simulink model "DiagCCaller_TestHarness"  (R2019a)
settings: Solver=FixedStepDiscrete  StartTime=0.0  StopTime=10.0  FixedStep=0.1  RelTol=1e-3  EnableMultiTasking=on
undefined symbols (not defined in the file): Dem_EventStatusType, sigbuilder_block
(part 3 of 4)

== system DiagCCaller_TestHarness/Fault set and recover , FaultCnt = 10, PassCnt = -5 , Heal =1, JumpDownEn = 0  ==
  Bus Creator : BusCreator  Inputs=15
  Data Type Conversion{,1..2,9..14} (9 alike) : DataTypeConversion  OutDataTypeStr=boolean
  Data Type Conversion3 : DataTypeConversion  OutDataTypeStr=single
  Data Type Conversion4 : DataTypeConversion  OutDataTypeStr=single
  Data Type Conversion{5..8} (4 alike) : DataTypeConversion  OutDataTypeStr=int16
  Signal Builder : Subsystem  Tag=STV Subsys  LoadFcn=sigbuilder_block('load');  StartFcn=sigbuilder_block('start');  StopFcn=sigbuilder_block('stop');  ClipboardFcn=sigbuilder_block('clipboard');  TreatAsAtomicUnit=on  mask(Sigbuilder block){tuvar=[0:10]}
      mask help: Simulink:masks:SigbuilderBlock_MD
      mask init:
      | if ~strcmp(get_param(bdroot(gcbh),'SimulationStatus'),'stopped') tuvar = sigbuilder_block('maskInit'); end
      settings: CopyFcn=sigbuilder_block('copy');  DeleteFcn=sigbuilder_block('delete');  ModelCloseFcn=sigbuilder_block('modelClose');  PreSaveFcn=sigbuilder_block('preSave');  PauseFcn=sigbuilder_block('pause');  ContinueFcn=sigbuilder_block('continue');  NameChangeFcn=sigbuilder_block('namechange');  OpenFcn=sigbuilder_block('open',[5.4 30 1141.2 522.6 ]);  CloseFcn=sigbuilder_block('close');
      mask Display: plot(0, 0, 100, 100,[2, 2, 32, 32, 2], [68, 8, 8, 68, 68],[32, 2], [38, 38], [32, 19, 2],[53, 60, 44], [32, 17, 17, 2],[16, 16, 31, 31]);txt = getActiveGroup(gcbh);text(2, 100, txt,'verticalAlignment', 'top');
  Out1 : Outport
  wires:
  Bus Creator/1 -> Out1/1
  Signal Builder/2(DiagInput) -> Data Type Conversion1/1
  Signal Builder/3(StartupComp) -> Data Type Conversion2/1
  Signal Builder/4(MaxValue) -> Data Type Conversion4/1
  Signal Builder/5(MinValue) -> Data Type Conversion3/1
  Signal Builder/6(UpCount) -> Data Type Conversion5/1
  Signal Builder/7(DownCount) -> Data Type Conversion6/1
  Signal Builder/8(FaultCountThd) -> Data Type Conversion7/1
  Signal Builder/9(PassCountThd) -> Data Type Conversion8/1
  Signal Builder/10(DebounceEn) -> Data Type Conversion9/1
  Signal Builder/11(DiagReset) -> Data Type Conversion10/1
  Signal Builder/12(DiagEnable) -> Data Type Conversion11/1
  Signal Builder/13(HealEnable) -> Data Type Conversion12/1
  Signal Builder/14(PreestorageFreezeTrigger) -> Data Type Conversion13/1
  Signal Builder/15(JumpDownEn) -> Data Type Conversion14/1
  Signal Builder/1(EnableSubsystem) -> Data Type Conversion/1
  Data Type Conversion/1 -> Bus Creator/1  "EnableSubsystem"
  Data Type Conversion1/1 -> Bus Creator/2  "DiagInput"
  Data Type Conversion2/1 -> Bus Creator/3  "StartupComp"
  Data Type Conversion4/1 -> Bus Creator/4  "MaxValue"
  Data Type Conversion3/1 -> Bus Creator/5  "MinValue"
  Data Type Conversion5/1 -> Bus Creator/6  "UpCount"
  Data Type Conversion6/1 -> Bus Creator/7  "DownCount"
  Data Type Conversion7/1 -> Bus Creator/8  "FaultCountThd"
  Data Type Conversion8/1 -> Bus Creator/9  "PassCountThd"
  Data Type Conversion9/1 -> Bus Creator/10  "DebounceEn"
  Data Type Conversion10/1 -> Bus Creator/11  "DiagReset"
  Data Type Conversion11/1 -> Bus Creator/12  "DiagEnable"
  Data Type Conversion12/1 -> Bus Creator/13  "HealEnable"
  Data Type Conversion13/1 -> Bus Creator/14  "PreestorageFreezeTrigger"
  Data Type Conversion14/1 -> Bus Creator/15  "JumpDownEn"

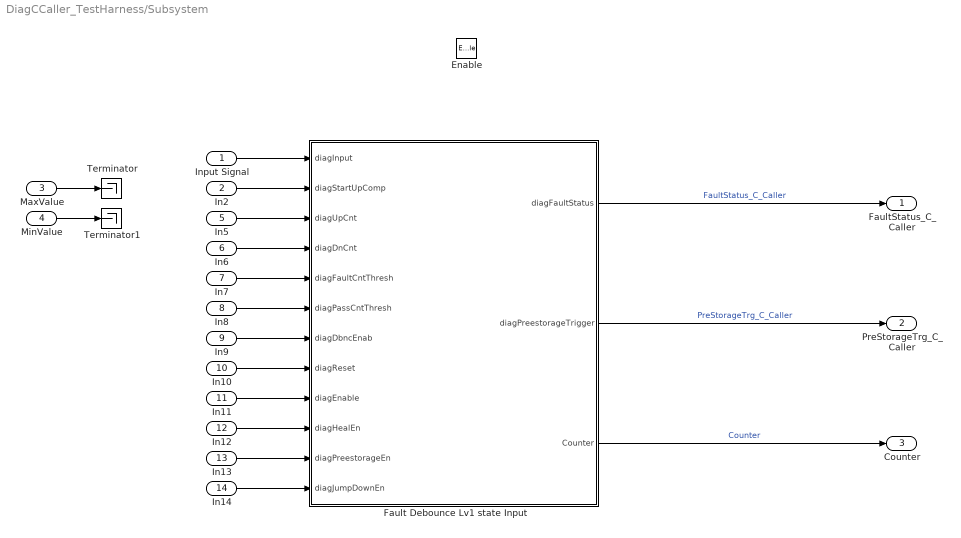
== system DiagCCaller_TestHarness/Subsystem ==
  Input Signal : Inport
  In2 : Inport  Port=2
  MaxValue : Inport  Port=3
  MinValue : Inport  Port=4
  In5 : Inport  Port=5
  In6 : Inport  Port=6
  In7 : Inport  Port=7
  In8 : Inport  Port=8
  In9 : Inport  Port=9
  In10 : Inport  Port=10
  In11 : Inport  Port=11
  In12 : Inport  Port=12
  In13 : Inport  Port=13
  In14 : Inport  Port=14
  Enable : EnablePort  StatesWhenEnabling=reset
  Fault Debounce Lv1 state Input : Subsystem  AncestorBlock=common_lib/Diagnostics/Fault Debounce Lv1 state Input
  Terminator : Terminator
  Terminator1 : Terminator
  FaultStatus_C_Caller : Outport
  PreStorageTrg_C_Caller : Outport  Port=2  OutputWhenDisabled=reset  InitialOutput=false
  Counter : Outport  Port=3
  wires:
  In2/1 -> Fault Debounce Lv1 state Input/2(diagStartUpComp)
  Fault Debounce Lv1 state Input/1(diagFaultStatus) -> FaultStatus_C_Caller/1  "FaultStatus_C_Caller"
  Input Signal/1 -> Fault Debounce Lv1 state Input/1(diagInput)
  Fault Debounce Lv1 state Input/2(diagPreestorageTrigger) -> PreStorageTrg_C_Caller/1  "PreStorageTrg_C_Caller"
  In7/1 -> Fault Debounce Lv1 state Input/5(diagFaultCntThresh)
  In12/1 -> Fault Debounce Lv1 state Input/10(diagHealEn)
  In6/1 -> Fault Debounce Lv1 state Input/4(diagDnCnt)
  In8/1 -> Fault Debounce Lv1 state Input/6(diagPassCntThresh)
  In14/1 -> Fault Debounce Lv1 state Input/12(diagJumpDownEn)
  In9/1 -> Fault Debounce Lv1 state Input/7(diagDbncEnab)
  In5/1 -> Fault Debounce Lv1 state Input/3(diagUpCnt)
  In11/1 -> Fault Debounce Lv1 state Input/9(diagEnable)
  In10/1 -> Fault Debounce Lv1 state Input/8(diagReset)
  In13/1 -> Fault Debounce Lv1 state Input/11(diagPreestorageEn)
  Fault Debounce Lv1 state Input/3(Counter) -> Counter/1  "Counter"
  MaxValue/1 -> Terminator/1
  MinValue/1 -> Terminator1/1

== system DiagCCaller_TestHarness/Debounce Enabled - Fault bounces , FaultCnt = 10, PassCnt = -5 , Heal =1, JumpDownEn = 1 /Signal Builder ==
  Demux : Demux  Tag=STV Demux  Outputs=15
  FromWs : FromWorkspace  Tag=STV FromWs  VariableName=tuvar  SampleTime=0
      SigBuilderData=|
      | common.afterFinalStr = 'Extrapolate'
      | common.sampleTime = 0
      | dataSet.timeRange = [0 10]
      | dataSet.name = 'Group 1'
      | sbobj.Groups.Name = 'Group 1'
      | sbobj.Groups.Signals(1).Name = 'EnableSubsystem'
      | sbobj.Groups.Signals(1).XData = [0 4.36 4.94 9.06 9.06 10]
      | sbobj.Groups.Signals(1).YData = [1 1 1 1 0 0]
      | sbobj.Groups.Signals(2).Name = 'DiagInput'
      | sbobj.Groups.Signals(2).XData = [0 1 1 3.03 3.03 4.6 4.6 5.3 5.3 5.7 5.7 6.4 6.4 6.7 6.7 7.3 7.3 7.7 7.7 8.35 8.35 10]
      | sbobj.Groups.Signals(2).YData = [0 0 1.1 1.1 0 0 1 1 0 0 1 1 0 0 1 1 0 0 1 1 0 0]
      | sbobj.Groups.Signals(3).Name = 'StartupComp'
      | sbobj.Groups.Signals(3).XData = [0 10]
      | sbobj.Groups.Signals(3).YData = [1 1]
      | sbobj.Groups.Signals(4).Name = 'MaxValue'
      | sbobj.Groups.Signals(4).XData = [0 10]
      | sbobj.Groups.Signals(4).YData = [9999 9999]
      | sbobj.Groups.Signals(5).Name = 'MinValue'
      | sbobj.Groups.Signals(5).XData = [0 10]
      | sbobj.Groups.Signals(5).YData = [-69.9 -69.9]
      | sbobj.Groups.Signals(6).Name = 'UpCount'
      | sbobj.Groups.Signals(6).XData = [0 10]
      | sbobj.Groups.Signals(6).YData = [1 1]
      | sbobj.Groups.Signals(7).Name = 'DownCount'
      | sbobj.Groups.Signals(7).XData = [0 10]
      | sbobj.Groups.Signals(7).YData = [1 1]
      | sbobj.Groups.Signals(8).Name = 'FaultCountThd'
      | sbobj.Groups.Signals(8).XData = [0 10]
      | sbobj.Groups.Signals(8).YData = [10 10]
      | sbobj.Groups.Signals(9).Name = 'PassCountThd'
      | sbobj.Groups.Signals(9).XData = [0 10]
      | sbobj.Groups.Signals(9).YData = [-5 -5]
      | sbobj.Groups.Signals(10).Name = 'DebounceEn'
      | sbobj.Groups.Signals(10).XData = [0 10]
      | sbobj.Groups.Signals(10).YData = [1 1]
      | sbobj.Groups.Signals(11).Name = 'DiagReset'
      | sbobj.Groups.Signals(11).XData = [0 10]
      | sbobj.Groups.Signals(11).YData = [0 0]
      | sbobj.Groups.Signals(12).Name = 'DiagEnable'
      | sbobj.Groups.Signals(12).XData = [0 10]
      | sbobj.Groups.Signals(12).YData = [1 1]
      | sbobj.Groups.Signals(13).Name = 'HealEnable'
      | sbobj.Groups.Signals(13).XData = [0 10]
      | sbobj.Groups.Signals(13).YData = [1 1]
      | sbobj.Groups.Signals(14).Name = 'PreestorageFreezeTrigger'
      | sbobj.Groups.Signals(14).XData = [0 10]
      | sbobj.Groups.Signals(14).YData = [1 1]
      | sbobj.Groups.Signals(15).Name = 'JumpDownEn'
      | sbobj.Groups.Signals(15).XData = [0 10]
      | sbobj.Groups.Signals(15).YData = [1 1]
  EnableSubsystem : Outport  Tag=STV Outport
  DiagInput : Outport  Tag=STV Outport  Port=2
  StartupComp : Outport  Tag=STV Outport  Port=3
  MaxValue : Outport  Tag=STV Outport  Port=4
  MinValue : Outport  Tag=STV Outport  Port=5
  UpCount : Outport  Tag=STV Outport  Port=6
  DownCount : Outport  Tag=STV Outport  Port=7
  FaultCountThd : Outport  Tag=STV Outport  Port=8
  PassCountThd : Outport  Tag=STV Outport  Port=9
  DebounceEn : Outport  Tag=STV Outport  Port=10
  DiagReset : Outport  Tag=STV Outport  Port=11
  DiagEnable : Outport  Tag=STV Outport  Port=12
  HealEnable : Outport  Tag=STV Outport  Port=13
  PreestorageFreezeTrigger : Outport  Tag=STV Outport  Port=14
  JumpDownEn : Outport  Tag=STV Outport  Port=15
  wires:
  FromWs/1 -> Demux/1
  Demux/1 -> EnableSubsystem/1
  Demux/2 -> DiagInput/1
  Demux/3 -> StartupComp/1
  Demux/4 -> MaxValue/1
  Demux/5 -> MinValue/1
  Demux/6 -> UpCount/1
  Demux/7 -> DownCount/1
  Demux/8 -> FaultCountThd/1
  Demux/9 -> PassCountThd/1
  Demux/10 -> DebounceEn/1
  Demux/11 -> DiagReset/1
  Demux/12 -> DiagEnable/1
  Demux/13 -> HealEnable/1
  Demux/14 -> PreestorageFreezeTrigger/1
  Demux/15 -> JumpDownEn/1

== system DiagCCaller_TestHarness/Debounce Enabled - Fault set and recover , FaultCnt = 10, PassCnt = -5 , Heal =1, JumpDownEn = 1 /Signal Builder ==
  Demux : Demux  Tag=STV Demux  Outputs=15
  FromWs : FromWorkspace  Tag=STV FromWs  VariableName=tuvar  SampleTime=0
      SigBuilderData=|
      | common.afterFinalStr = 'Extrapolate'
      | common.sampleTime = 0
      | dataSet.timeRange = [0 10]
      | dataSet.name = 'Group 1'
      | sbobj.Groups.Name = 'Group 1'
      | sbobj.Groups.Signals(1).Name = 'EnableSubsystem'
      | sbobj.Groups.Signals(1).XData = [0 4.36 4.94 9.06 9.06 10]
      | sbobj.Groups.Signals(1).YData = [1 1 1 1 0 0]
      | sbobj.Groups.Signals(2).Name = 'DiagInput'
      | sbobj.Groups.Signals(2).XData = [0 1 1 3.03 3.03 4.91 4.91 6.65 6.65 10]
      | sbobj.Groups.Signals(2).YData = [0 0 1.1 1.1 0 0 1.2 1.2 0 0]
      | sbobj.Groups.Signals(3).Name = 'StartupComp'
      | sbobj.Groups.Signals(3).XData = [0 10]
      | sbobj.Groups.Signals(3).YData = [1 1]
      | sbobj.Groups.Signals(4).Name = 'MaxValue'
      | sbobj.Groups.Signals(4).XData = [0 10]
      | sbobj.Groups.Signals(4).YData = [9999 9999]
      | sbobj.Groups.Signals(5).Name = 'MinValue'
      | sbobj.Groups.Signals(5).XData = [0 10]
      | sbobj.Groups.Signals(5).YData = [-69.9 -69.9]
      | sbobj.Groups.Signals(6).Name = 'UpCount'
      | sbobj.Groups.Signals(6).XData = [0 10]
      | sbobj.Groups.Signals(6).YData = [1 1]
      | sbobj.Groups.Signals(7).Name = 'DownCount'
      | sbobj.Groups.Signals(7).XData = [0 10]
      | sbobj.Groups.Signals(7).YData = [1 1]
      | sbobj.Groups.Signals(8).Name = 'FaultCountThd'
      | sbobj.Groups.Signals(8).XData = [0 10]
      | sbobj.Groups.Signals(8).YData = [10 10]
      | sbobj.Groups.Signals(9).Name = 'PassCountThd'
      | sbobj.Groups.Signals(9).XData = [0 10]
      | sbobj.Groups.Signals(9).YData = [-5 -5]
      | sbobj.Groups.Signals(10).Name = 'DebounceEn'
      | sbobj.Groups.Signals(10).XData = [0 10]
      | sbobj.Groups.Signals(10).YData = [1 1]
      | sbobj.Groups.Signals(11).Name = 'DiagReset'
      | sbobj.Groups.Signals(11).XData = [0 10]
      | sbobj.Groups.Signals(11).YData = [0 0]
      | sbobj.Groups.Signals(12).Name = 'DiagEnable'
      | sbobj.Groups.Signals(12).XData = [0 10]
      | sbobj.Groups.Signals(12).YData = [1 1]
      | sbobj.Groups.Signals(13).Name = 'HealEnable'
      | sbobj.Groups.Signals(13).XData = [0 10]
      | sbobj.Groups.Signals(13).YData = [1 1]
      | sbobj.Groups.Signals(14).Name = 'PreestorageFreezeTrigger'
      | sbobj.Groups.Signals(14).XData = [0 10]
      | sbobj.Groups.Signals(14).YData = [1 1]
      | sbobj.Groups.Signals(15).Name = 'JumpDownEn'
      | sbobj.Groups.Signals(15).XData = [0 10]
      | sbobj.Groups.Signals(15).YData = [1 1]
  EnableSubsystem : Outport  Tag=STV Outport
  DiagInput : Outport  Tag=STV Outport  Port=2
  StartupComp : Outport  Tag=STV Outport  Port=3
  MaxValue : Outport  Tag=STV Outport  Port=4
  MinValue : Outport  Tag=STV Outport  Port=5
  UpCount : Outport  Tag=STV Outport  Port=6
  DownCount : Outport  Tag=STV Outport  Port=7
  FaultCountThd : Outport  Tag=STV Outport  Port=8
  PassCountThd : Outport  Tag=STV Outport  Port=9
  DebounceEn : Outport  Tag=STV Outport  Port=10
  DiagReset : Outport  Tag=STV Outport  Port=11
  DiagEnable : Outport  Tag=STV Outport  Port=12
  HealEnable : Outport  Tag=STV Outport  Port=13
  PreestorageFreezeTrigger : Outport  Tag=STV Outport  Port=14
  JumpDownEn : Outport  Tag=STV Outport  Port=15
  wires:
  Demux/15 -> JumpDownEn/1
  Demux/14 -> PreestorageFreezeTrigger/1
  Demux/13 -> HealEnable/1
  Demux/12 -> DiagEnable/1
  Demux/11 -> DiagReset/1
  Demux/10 -> DebounceEn/1
  Demux/9 -> PassCountThd/1
  Demux/8 -> FaultCountThd/1
  Demux/7 -> DownCount/1
  Demux/6 -> UpCount/1
  Demux/5 -> MinValue/1
  Demux/4 -> MaxValue/1
  Demux/3 -> StartupComp/1
  Demux/2 -> DiagInput/1
  Demux/1 -> EnableSubsystem/1
  FromWs/1 -> Demux/1

== system DiagCCaller_TestHarness/Debounce Enabled - Fault set and recover , FaultCnt = 10, PassCnt = 0 , Heal =0, JumpDownEn = 0 /Signal Builder ==
  Demux : Demux  Tag=STV Demux  Outputs=15
  FromWs : FromWorkspace  Tag=STV FromWs  VariableName=tuvar  SampleTime=0
      SigBuilderData=|
      | common.afterFinalStr = 'Extrapolate'
      | common.sampleTime = 0
      | dataSet.timeRange = [0 10]
      | dataSet.name = 'Group 1'
      | sbobj.Groups.Name = 'Group 1'
      | sbobj.Groups.Signals(1).Name = 'EnableSubsystem'
      | sbobj.Groups.Signals(1).XData = [0 4.36 4.94 9.06 9.06 10]
      | sbobj.Groups.Signals(1).YData = [1 1 1 1 0 0]
      | sbobj.Groups.Signals(2).Name = 'DiagInput'
      | sbobj.Groups.Signals(2).XData = [0 1 1 2.75 2.75 4.59 4.59 6.52 6.52 10]
      | sbobj.Groups.Signals(2).YData = [0 0 1.1 1.1 0 0 1.2 1.2 0 0]
      | sbobj.Groups.Signals(3).Name = 'StartupComp'
      | sbobj.Groups.Signals(3).XData = [0 10]
      | sbobj.Groups.Signals(3).YData = [1 1]
      | sbobj.Groups.Signals(4).Name = 'MaxValue'
      | sbobj.Groups.Signals(4).XData = [0 10]
      | sbobj.Groups.Signals(4).YData = [9999 9999]
      | sbobj.Groups.Signals(5).Name = 'MinValue'
      | sbobj.Groups.Signals(5).XData = [0 10]
      | sbobj.Groups.Signals(5).YData = [-69.9 -69.9]
      | sbobj.Groups.Signals(6).Name = 'UpCount'
      | sbobj.Groups.Signals(6).XData = [0 10]
      | sbobj.Groups.Signals(6).YData = [1 1]
      | sbobj.Groups.Signals(7).Name = 'DownCount'
      | sbobj.Groups.Signals(7).XData = [0 10]
      | sbobj.Groups.Signals(7).YData = [1 1]
      | sbobj.Groups.Signals(8).Name = 'FaultCountThd'
      | sbobj.Groups.Signals(8).XData = [0 10]
      | sbobj.Groups.Signals(8).YData = [10 10]
      | sbobj.Groups.Signals(9).Name = 'PassCountThd'
      | sbobj.Groups.Signals(9).XData = [0 10]
      | sbobj.Groups.Signals(9).YData = [0 0]
      | sbobj.Groups.Signals(10).Name = 'DebounceEn'
      | sbobj.Groups.Signals(10).XData = [0 10]
      | sbobj.Groups.Signals(10).YData = [1 1]
      | sbobj.Groups.Signals(11).Name = 'DiagReset'
      | sbobj.Groups.Signals(11).XData = [0 10]
      | sbobj.Groups.Signals(11).YData = [0 0]
      | sbobj.Groups.Signals(12).Name = 'DiagEnable'
      | sbobj.Groups.Signals(12).XData = [0 10]
      | sbobj.Groups.Signals(12).YData = [1 1]
      | sbobj.Groups.Signals(13).Name = 'HealEnable'
      | sbobj.Groups.Signals(13).XData = [0 10]
      | sbobj.Groups.Signals(13).YData = [0 0]
      | sbobj.Groups.Signals(14).Name = 'PreestorageFreezeTrigger'
      | sbobj.Groups.Signals(14).XData = [0 10]
      | sbobj.Groups.Signals(14).YData = [1 1]
      | sbobj.Groups.Signals(15).Name = 'JumpDownEn'
      | sbobj.Groups.Signals(15).XData = [0 10]
      | sbobj.Groups.Signals(15).YData = [0 0]
  EnableSubsystem : Outport  Tag=STV Outport
  DiagInput : Outport  Tag=STV Outport  Port=2
  StartupComp : Outport  Tag=STV Outport  Port=3
  MaxValue : Outport  Tag=STV Outport  Port=4
  MinValue : Outport  Tag=STV Outport  Port=5
  UpCount : Outport  Tag=STV Outport  Port=6
  DownCount : Outport  Tag=STV Outport  Port=7
  FaultCountThd : Outport  Tag=STV Outport  Port=8
  PassCountThd : Outport  Tag=STV Outport  Port=9
  DebounceEn : Outport  Tag=STV Outport  Port=10
  DiagReset : Outport  Tag=STV Outport  Port=11
  DiagEnable : Outport  Tag=STV Outport  Port=12
  HealEnable : Outport  Tag=STV Outport  Port=13
  PreestorageFreezeTrigger : Outport  Tag=STV Outport  Port=14
  JumpDownEn : Outport  Tag=STV Outport  Port=15
  wires:
  Demux/15 -> JumpDownEn/1
  Demux/14 -> PreestorageFreezeTrigger/1
  Demux/13 -> HealEnable/1
  Demux/12 -> DiagEnable/1
  Demux/11 -> DiagReset/1
  Demux/10 -> DebounceEn/1
  Demux/9 -> PassCountThd/1
  Demux/8 -> FaultCountThd/1
  Demux/7 -> DownCount/1
  Demux/6 -> UpCount/1
  Demux/5 -> MinValue/1
  Demux/4 -> MaxValue/1
  Demux/3 -> StartupComp/1
  Demux/2 -> DiagInput/1
  Demux/1 -> EnableSubsystem/1
  FromWs/1 -> Demux/1

== system DiagCCaller_TestHarness/Debounce Enabled - Fault set and recover , FaultCnt = 10, PassCnt = 0 , Heal =0, JumpDownEn = 1 /Signal Builder ==
  Demux : Demux  Tag=STV Demux  Outputs=15
  FromWs : FromWorkspace  Tag=STV FromWs  VariableName=tuvar  SampleTime=0
      SigBuilderData=|
      | common.afterFinalStr = 'Extrapolate'
      | common.sampleTime = 0
      | dataSet.timeRange = [0 10]
      | dataSet.name = 'Group 1'
      | sbobj.Groups.Name = 'Group 1'
      | sbobj.Groups.Signals(1).Name = 'EnableSubsystem'
      | sbobj.Groups.Signals(1).XData = [0 4.36 4.94 9.06 9.06 10]
      | sbobj.Groups.Signals(1).YData = [1 1 1 1 0 0]
      | sbobj.Groups.Signals(2).Name = 'DiagInput'
      | sbobj.Groups.Signals(2).XData = [0 1 1 3.03 3.03 4.91 4.91 6.65 6.65 10]
      | sbobj.Groups.Signals(2).YData = [0 0 1.1 1.1 0 0 1.2 1.2 0 0]
      | sbobj.Groups.Signals(3).Name = 'StartupComp'
      | sbobj.Groups.Signals(3).XData = [0 10]
      | sbobj.Groups.Signals(3).YData = [1 1]
      | sbobj.Groups.Signals(4).Name = 'MaxValue'
      | sbobj.Groups.Signals(4).XData = [0 10]
      | sbobj.Groups.Signals(4).YData = [9999 9999]
      | sbobj.Groups.Signals(5).Name = 'MinValue'
      | sbobj.Groups.Signals(5).XData = [0 10]
      | sbobj.Groups.Signals(5).YData = [-69.9 -69.9]
      | sbobj.Groups.Signals(6).Name = 'UpCount'
      | sbobj.Groups.Signals(6).XData = [0 10]
      | sbobj.Groups.Signals(6).YData = [1 1]
      | sbobj.Groups.Signals(7).Name = 'DownCount'
      | sbobj.Groups.Signals(7).XData = [0 10]
      | sbobj.Groups.Signals(7).YData = [1 1]
      | sbobj.Groups.Signals(8).Name = 'FaultCountThd'
      | sbobj.Groups.Signals(8).XData = [0 10]
      | sbobj.Groups.Signals(8).YData = [10 10]
      | sbobj.Groups.Signals(9).Name = 'PassCountThd'
      | sbobj.Groups.Signals(9).XData = [0 10]
      | sbobj.Groups.Signals(9).YData = [0 0]
      | sbobj.Groups.Signals(10).Name = 'DebounceEn'
      | sbobj.Groups.Signals(10).XData = [0 10]
      | sbobj.Groups.Signals(10).YData = [1 1]
      | sbobj.Groups.Signals(11).Name = 'DiagReset'
      | sbobj.Groups.Signals(11).XData = [0 10]
      | sbobj.Groups.Signals(11).YData = [0 0]
      | sbobj.Groups.Signals(12).Name = 'DiagEnable'
      | sbobj.Groups.Signals(12).XData = [0 10]
      | sbobj.Groups.Signals(12).YData = [1 1]
      | sbobj.Groups.Signals(13).Name = 'HealEnable'
      | sbobj.Groups.Signals(13).XData = [0 10]
      | sbobj.Groups.Signals(13).YData = [0 0]
      | sbobj.Groups.Signals(14).Name = 'PreestorageFreezeTrigger'
      | sbobj.Groups.Signals(14).XData = [0 10]
      | sbobj.Groups.Signals(14).YData = [1 1]
      | sbobj.Groups.Signals(15).Name = 'JumpDownEn'
      | sbobj.Groups.Signals(15).XData = [0 10]
      | sbobj.Groups.Signals(15).YData = [1 1]
  EnableSubsystem : Outport  Tag=STV Outport
  DiagInput : Outport  Tag=STV Outport  Port=2
  StartupComp : Outport  Tag=STV Outport  Port=3
  MaxValue : Outport  Tag=STV Outport  Port=4
  MinValue : Outport  Tag=STV Outport  Port=5
  UpCount : Outport  Tag=STV Outport  Port=6
  DownCount : Outport  Tag=STV Outport  Port=7
  FaultCountThd : Outport  Tag=STV Outport  Port=8
  PassCountThd : Outport  Tag=STV Outport  Port=9
  DebounceEn : Outport  Tag=STV Outport  Port=10
  DiagReset : Outport  Tag=STV Outport  Port=11
  DiagEnable : Outport  Tag=STV Outport  Port=12
  HealEnable : Outport  Tag=STV Outport  Port=13
  PreestorageFreezeTrigger : Outport  Tag=STV Outport  Port=14
  JumpDownEn : Outport  Tag=STV Outport  Port=15
  wires:
  FromWs/1 -> Demux/1
  Demux/1 -> EnableSubsystem/1
  Demux/2 -> DiagInput/1
  Demux/3 -> StartupComp/1
  Demux/4 -> MaxValue/1
  Demux/5 -> MinValue/1
  Demux/6 -> UpCount/1
  Demux/7 -> DownCount/1
  Demux/8 -> FaultCountThd/1
  Demux/9 -> PassCountThd/1
  Demux/10 -> DebounceEn/1
  Demux/11 -> DiagReset/1
  Demux/12 -> DiagEnable/1
  Demux/13 -> HealEnable/1
  Demux/14 -> PreestorageFreezeTrigger/1
  Demux/15 -> JumpDownEn/1

== system DiagCCaller_TestHarness/Debounce Enabled - INIT Fault Active , FaultCnt = 10, PassCnt = -5 , Heal 1 /Signal Builder ==
  Demux : Demux  Tag=STV Demux  Outputs=15
  FromWs : FromWorkspace  Tag=STV FromWs  VariableName=tuvar  SampleTime=0
      SigBuilderData=|
      | common.afterFinalStr = 'Extrapolate'
      | common.sampleTime = 0
      | dataSet.timeRange = [0 10]
      | dataSet.name = 'Group 1'
      | sbobj.Groups.Name = 'Group 1'
      | sbobj.Groups.Signals(1).Name = 'EnableSubsystem'
      | sbobj.Groups.Signals(1).XData = [0 4.36 4.94 9.06 9.06 10]
      | sbobj.Groups.Signals(1).YData = [1 1 1 1 0 0]
      | sbobj.Groups.Signals(2).Name = 'DiagInput'
      | sbobj.Groups.Signals(2).XData = [0 1.7 1.7 2.41 3.88 3.88 6 6 8 8 9.5 9.5 10]
      | sbobj.Groups.Signals(2).YData = [1 1 0 0 0 1.1 1.1 0 0 1.2 1.2 0 0]
      | sbobj.Groups.Signals(3).Name = 'StartupComp'
      | sbobj.Groups.Signals(3).XData = [0 10]
      | sbobj.Groups.Signals(3).YData = [1 1]
      | sbobj.Groups.Signals(4).Name = 'MaxValue'
      | sbobj.Groups.Signals(4).XData = [0 10]
      | sbobj.Groups.Signals(4).YData = [9999 9999]
      | sbobj.Groups.Signals(5).Name = 'MinValue'
      | sbobj.Groups.Signals(5).XData = [0 10]
      | sbobj.Groups.Signals(5).YData = [-69.9 -69.9]
      | sbobj.Groups.Signals(6).Name = 'UpCount'
      | sbobj.Groups.Signals(6).XData = [0 10]
      | sbobj.Groups.Signals(6).YData = [1 1]
      | sbobj.Groups.Signals(7).Name = 'DownCount'
      | sbobj.Groups.Signals(7).XData = [0 10]
      | sbobj.Groups.Signals(7).YData = [1 1]
      | sbobj.Groups.Signals(8).Name = 'FaultCountThd'
      | sbobj.Groups.Signals(8).XData = [0 10]
      | sbobj.Groups.Signals(8).YData = [10 10]
      | sbobj.Groups.Signals(9).Name = 'PassCountThd'
      | sbobj.Groups.Signals(9).XData = [0 10]
      | sbobj.Groups.Signals(9).YData = [-5 -5]
      | sbobj.Groups.Signals(10).Name = 'DebounceEn'
      | sbobj.Groups.Signals(10).XData = [0 10]
      | sbobj.Groups.Signals(10).YData = [1 1]
      | sbobj.Groups.Signals(11).Name = 'DiagReset'
      | sbobj.Groups.Signals(11).XData = [0 10]
      | sbobj.Groups.Signals(11).YData = [0 0]
      | sbobj.Groups.Signals(12).Name = 'DiagEnable'
      | sbobj.Groups.Signals(12).XData = [0 10]
      | sbobj.Groups.Signals(12).YData = [1 1]
      | sbobj.Groups.Signals(13).Name = 'HealEnable'
      | sbobj.Groups.Signals(13).XData = [0 10]
      | sbobj.Groups.Signals(13).YData = [1 1]
      | sbobj.Groups.Signals(14).Name = 'PreestorageFreezeTrigger'
      | sbobj.Groups.Signals(14).XData = [0 10]
      | sbobj.Groups.Signals(14).YData = [1 1]
      | sbobj.Groups.Signals(15).Name = 'JumpDownEn'
      | sbobj.Groups.Signals(15).XData = [0 10]
      | sbobj.Groups.Signals(15).YData = [0 0]
  EnableSubsystem : Outport  Tag=STV Outport
  DiagInput : Outport  Tag=STV Outport  Port=2
  StartupComp : Outport  Tag=STV Outport  Port=3
  MaxValue : Outport  Tag=STV Outport  Port=4
  MinValue : Outport  Tag=STV Outport  Port=5
  UpCount : Outport  Tag=STV Outport  Port=6
  DownCount : Outport  Tag=STV Outport  Port=7
  FaultCountThd : Outport  Tag=STV Outport  Port=8
  PassCountThd : Outport  Tag=STV Outport  Port=9
  DebounceEn : Outport  Tag=STV Outport  Port=10
  DiagReset : Outport  Tag=STV Outport  Port=11
  DiagEnable : Outport  Tag=STV Outport  Port=12
  HealEnable : Outport  Tag=STV Outport  Port=13
  PreestorageFreezeTrigger : Outport  Tag=STV Outport  Port=14
  JumpDownEn : Outport  Tag=STV Outport  Port=15
  wires:
  Demux/15 -> JumpDownEn/1
  Demux/14 -> PreestorageFreezeTrigger/1
  Demux/13 -> HealEnable/1
  Demux/12 -> DiagEnable/1
  Demux/11 -> DiagReset/1
  Demux/10 -> DebounceEn/1
  Demux/9 -> PassCountThd/1
  Demux/8 -> FaultCountThd/1
  Demux/7 -> DownCount/1
  Demux/6 -> UpCount/1
  Demux/5 -> MinValue/1
  Demux/4 -> MaxValue/1
  Demux/3 -> StartupComp/1
  Demux/2 -> DiagInput/1
  Demux/1 -> EnableSubsystem/1
  FromWs/1 -> Demux/1

== system DiagCCaller_TestHarness/Debounce Enabled - INIT Fault Active , FaultCnt = 10, PassCnt = 0 , Heal 0 /Signal Builder ==
  Demux : Demux  Tag=STV Demux  Outputs=15
  FromWs : FromWorkspace  Tag=STV FromWs  VariableName=tuvar  SampleTime=0
      SigBuilderData=|
      | common.afterFinalStr = 'Extrapolate'
      | common.sampleTime = 0
      | dataSet.timeRange = [0 10]
      | dataSet.name = 'Group 1'
      | sbobj.Groups.Name = 'Group 1'
      | sbobj.Groups.Signals(1).Name = 'EnableSubsystem'
      | sbobj.Groups.Signals(1).XData = [0 4.36 4.94 9.06 9.06 10]
      | sbobj.Groups.Signals(1).YData = [1 1 1 1 0 0]
      | sbobj.Groups.Signals(2).Name = 'DiagInput'
      | sbobj.Groups.Signals(2).XData = [0 1 2.41 2.41 4.96 4.96 6.69 6.69 8.36 8.36 9.5 9.5 10]
      | sbobj.Groups.Signals(2).YData = [1 1 1 0 0 1.1 1.1 0 0 1.2 1.2 0 0]
      | sbobj.Groups.Signals(3).Name = 'StartupComp'
      | sbobj.Groups.Signals(3).XData = [0 10]
      | sbobj.Groups.Signals(3).YData = [1 1]
      | sbobj.Groups.Signals(4).Name = 'MaxValue'
      | sbobj.Groups.Signals(4).XData = [0 10]
      | sbobj.Groups.Signals(4).YData = [9999 9999]
      | sbobj.Groups.Signals(5).Name = 'MinValue'
      | sbobj.Groups.Signals(5).XData = [0 10]
      | sbobj.Groups.Signals(5).YData = [-69.9 -69.9]
      | sbobj.Groups.Signals(6).Name = 'UpCount'
      | sbobj.Groups.Signals(6).XData = [0 10]
      | sbobj.Groups.Signals(6).YData = [1 1]
      | sbobj.Groups.Signals(7).Name = 'DownCount'
      | sbobj.Groups.Signals(7).XData = [0 10]
      | sbobj.Groups.Signals(7).YData = [1 1]
      | sbobj.Groups.Signals(8).Name = 'FaultCountThd'
      | sbobj.Groups.Signals(8).XData = [0 10]
      | sbobj.Groups.Signals(8).YData = [10 10]
      | sbobj.Groups.Signals(9).Name = 'PassCountThd'
      | sbobj.Groups.Signals(9).XData = [0 10]
      | sbobj.Groups.Signals(9).YData = [0 0]
      | sbobj.Groups.Signals(10).Name = 'DebounceEn'
      | sbobj.Groups.Signals(10).XData = [0 10]
      | sbobj.Groups.Signals(10).YData = [1 1]
      | sbobj.Groups.Signals(11).Name = 'DiagReset'
      | sbobj.Groups.Signals(11).XData = [0 10]
      | sbobj.Groups.Signals(11).YData = [0 0]
      | sbobj.Groups.Signals(12).Name = 'DiagEnable'
      | sbobj.Groups.Signals(12).XData = [0 10]
      | sbobj.Groups.Signals(12).YData = [1 1]
      | sbobj.Groups.Signals(13).Name = 'HealEnable'
      | sbobj.Groups.Signals(13).XData = [0 10]
      | sbobj.Groups.Signals(13).YData = [0 0]
      | sbobj.Groups.Signals(14).Name = 'PreestorageFreezeTrigger'
      | sbobj.Groups.Signals(14).XData = [0 10]
      | sbobj.Groups.Signals(14).YData = [1 1]
      | sbobj.Groups.Signals(15).Name = 'JumpDownEn'
      | sbobj.Groups.Signals(15).XData = [0 10]
      | sbobj.Groups.Signals(15).YData = [1 1]
  EnableSubsystem : Outport  Tag=STV Outport
  DiagInput : Outport  Tag=STV Outport  Port=2
  StartupComp : Outport  Tag=STV Outport  Port=3
  MaxValue : Outport  Tag=STV Outport  Port=4
  MinValue : Outport  Tag=STV Outport  Port=5
  UpCount : Outport  Tag=STV Outport  Port=6
  DownCount : Outport  Tag=STV Outport  Port=7
  FaultCountThd : Outport  Tag=STV Outport  Port=8
  PassCountThd : Outport  Tag=STV Outport  Port=9
  DebounceEn : Outport  Tag=STV Outport  Port=10
  DiagReset : Outport  Tag=STV Outport  Port=11
  DiagEnable : Outport  Tag=STV Outport  Port=12
  HealEnable : Outport  Tag=STV Outport  Port=13
  PreestorageFreezeTrigger : Outport  Tag=STV Outport  Port=14
  JumpDownEn : Outport  Tag=STV Outport  Port=15
  wires:
  Demux/15 -> JumpDownEn/1
  Demux/14 -> PreestorageFreezeTrigger/1
  Demux/13 -> HealEnable/1
  Demux/12 -> DiagEnable/1
  Demux/11 -> DiagReset/1
  Demux/10 -> DebounceEn/1
  Demux/9 -> PassCountThd/1
  Demux/8 -> FaultCountThd/1
  Demux/7 -> DownCount/1
  Demux/6 -> UpCount/1
  Demux/5 -> MinValue/1
  Demux/4 -> MaxValue/1
  Demux/3 -> StartupComp/1
  Demux/2 -> DiagInput/1
  Demux/1 -> EnableSubsystem/1
  FromWs/1 -> Demux/1

== system DiagCCaller_TestHarness/Debounce Enabled - INIT Fault Inactive , FaultCnt = 10, PassCnt = -5 , Heal 1 /Signal Builder ==
  Demux : Demux  Tag=STV Demux  Outputs=15
  FromWs : FromWorkspace  Tag=STV FromWs  VariableName=tuvar  SampleTime=0
      SigBuilderData=|
      | common.afterFinalStr = 'Extrapolate'
      | common.sampleTime = 0
      | dataSet.timeRange = [0 10]
      | dataSet.name = 'Group 1'
      | sbobj.Groups.Name = 'Group 1'
      | sbobj.Groups.Signals(1).Name = 'EnableSubsystem'
      | sbobj.Groups.Signals(1).XData = [0 4.36 4.94 9.06 9.06 10]
      | sbobj.Groups.Signals(1).YData = [1 1 1 1 0 0]
      | sbobj.Groups.Signals(2).Name = 'DiagInput'
      | sbobj.Groups.Signals(2).XData = [0 1 2.41 3.88 3.88 6 6 8 8 9.5 9.5 10]
      | sbobj.Groups.Signals(2).YData = [0 0 0 0 1.1 1.1 0 0 1.2 1.2 0 0]
      | sbobj.Groups.Signals(3).Name = 'StartupComp'
      | sbobj.Groups.Signals(3).XData = [0 10]
      | sbobj.Groups.Signals(3).YData = [1 1]
      | sbobj.Groups.Signals(4).Name = 'MaxValue'
      | sbobj.Groups.Signals(4).XData = [0 10]
      | sbobj.Groups.Signals(4).YData = [9999 9999]
      | sbobj.Groups.Signals(5).Name = 'MinValue'
      | sbobj.Groups.Signals(5).XData = [0 10]
      | sbobj.Groups.Signals(5).YData = [-69.9 -69.9]
      | sbobj.Groups.Signals(6).Name = 'UpCount'
      | sbobj.Groups.Signals(6).XData = [0 10]
      | sbobj.Groups.Signals(6).YData = [1 1]
      | sbobj.Groups.Signals(7).Name = 'DownCount'
      | sbobj.Groups.Signals(7).XData = [0 10]
      | sbobj.Groups.Signals(7).YData = [1 1]
      | sbobj.Groups.Signals(8).Name = 'FaultCountThd'
      | sbobj.Groups.Signals(8).XData = [0 10]
      | sbobj.Groups.Signals(8).YData = [10 10]
      | sbobj.Groups.Signals(9).Name = 'PassCountThd'
      | sbobj.Groups.Signals(9).XData = [0 10]
      | sbobj.Groups.Signals(9).YData = [-5 -5]
      | sbobj.Groups.Signals(10).Name = 'DebounceEn'
      | sbobj.Groups.Signals(10).XData = [0 10]
      | sbobj.Groups.Signals(10).YData = [1 1]
      | sbobj.Groups.Signals(11).Name = 'DiagReset'
      | sbobj.Groups.Signals(11).XData = [0 10]
      | sbobj.Groups.Signals(11).YData = [0 0]
      | sbobj.Groups.Signals(12).Name = 'DiagEnable'
      | sbobj.Groups.Signals(12).XData = [0 10]
      | sbobj.Groups.Signals(12).YData = [1 1]
      | sbobj.Groups.Signals(13).Name = 'HealEnable'
      | sbobj.Groups.Signals(13).XData = [0 10]
      | sbobj.Groups.Signals(13).YData = [1 1]
      | sbobj.Groups.Signals(14).Name = 'PreestorageFreezeTrigger'
      | sbobj.Groups.Signals(14).XData = [0 10]
      | sbobj.Groups.Signals(14).YData = [1 1]
      | sbobj.Groups.Signals(15).Name = 'JumpDownEn'
      | sbobj.Groups.Signals(15).XData = [0 10]
      | sbobj.Groups.Signals(15).YData = [0 0]
  EnableSubsystem : Outport  Tag=STV Outport
  DiagInput : Outport  Tag=STV Outport  Port=2
  StartupComp : Outport  Tag=STV Outport  Port=3
  MaxValue : Outport  Tag=STV Outport  Port=4
  MinValue : Outport  Tag=STV Outport  Port=5
  UpCount : Outport  Tag=STV Outport  Port=6
  DownCount : Outport  Tag=STV Outport  Port=7
  FaultCountThd : Outport  Tag=STV Outport  Port=8
  PassCountThd : Outport  Tag=STV Outport  Port=9
  DebounceEn : Outport  Tag=STV Outport  Port=10
  DiagReset : Outport  Tag=STV Outport  Port=11
  DiagEnable : Outport  Tag=STV Outport  Port=12
  HealEnable : Outport  Tag=STV Outport  Port=13
  PreestorageFreezeTrigger : Outport  Tag=STV Outport  Port=14
  JumpDownEn : Outport  Tag=STV Outport  Port=15
  wires:
  FromWs/1 -> Demux/1
  Demux/1 -> EnableSubsystem/1
  Demux/2 -> DiagInput/1
  Demux/3 -> StartupComp/1
  Demux/4 -> MaxValue/1
  Demux/5 -> MinValue/1
  Demux/6 -> UpCount/1
  Demux/7 -> DownCount/1
  Demux/8 -> FaultCountThd/1
  Demux/9 -> PassCountThd/1
  Demux/10 -> DebounceEn/1
  Demux/11 -> DiagReset/1
  Demux/12 -> DiagEnable/1
  Demux/13 -> HealEnable/1
  Demux/14 -> PreestorageFreezeTrigger/1
  Demux/15 -> JumpDownEn/1

== system DiagCCaller_TestHarness/Debounce Enabled - INIT Fault Inactive , FaultCnt = 10, PassCnt = 0 , Heal 0 /Signal Builder ==
  Demux : Demux  Tag=STV Demux  Outputs=15
  FromWs : FromWorkspace  Tag=STV FromWs  VariableName=tuvar  SampleTime=0
      SigBuilderData=|
      | common.afterFinalStr = 'Extrapolate'
      | common.sampleTime = 0
      | dataSet.timeRange = [0 10]
      | dataSet.name = 'Group 1'
      | sbobj.Groups.Name = 'Group 1'
      | sbobj.Groups.Signals(1).Name = 'EnableSubsystem'
      | sbobj.Groups.Signals(1).XData = [0 4.36 4.94 9.06 9.06 10]
      | sbobj.Groups.Signals(1).YData = [1 1 1 1 0 0]
      | sbobj.Groups.Signals(2).Name = 'DiagInput'
      | sbobj.Groups.Signals(2).XData = [0 1 2.41 3.88 3.88 6 6 8 8 9.5 9.5 10]
      | sbobj.Groups.Signals(2).YData = [0 0 0 0 1.1 1.1 0 0 1.2 1.2 0 0]
      | sbobj.Groups.Signals(3).Name = 'StartupComp'
      | sbobj.Groups.Signals(3).XData = [0 10]
      | sbobj.Groups.Signals(3).YData = [1 1]
      | sbobj.Groups.Signals(4).Name = 'MaxValue'
      | sbobj.Groups.Signals(4).XData = [0 10]
      | sbobj.Groups.Signals(4).YData = [9999 9999]
      | sbobj.Groups.Signals(5).Name = 'MinValue'
      | sbobj.Groups.Signals(5).XData = [0 10]
      | sbobj.Groups.Signals(5).YData = [-69.9 -69.9]
      | sbobj.Groups.Signals(6).Name = 'UpCount'
      | sbobj.Groups.Signals(6).XData = [0 10]
      | sbobj.Groups.Signals(6).YData = [1 1]
      | sbobj.Groups.Signals(7).Name = 'DownCount'
      | sbobj.Groups.Signals(7).XData = [0 10]
      | sbobj.Groups.Signals(7).YData = [1 1]
      | sbobj.Groups.Signals(8).Name = 'FaultCountThd'
      | sbobj.Groups.Signals(8).XData = [0 10]
      | sbobj.Groups.Signals(8).YData = [10 10]
      | sbobj.Groups.Signals(9).Name = 'PassCountThd'
      | sbobj.Groups.Signals(9).XData = [0 10]
      | sbobj.Groups.Signals(9).YData = [0 0]
      | sbobj.Groups.Signals(10).Name = 'DebounceEn'
      | sbobj.Groups.Signals(10).XData = [0 10]
      | sbobj.Groups.Signals(10).YData = [1 1]
      | sbobj.Groups.Signals(11).Name = 'DiagReset'
      | sbobj.Groups.Signals(11).XData = [0 10]
      | sbobj.Groups.Signals(11).YData = [0 0]
      | sbobj.Groups.Signals(12).Name = 'DiagEnable'
      | sbobj.Groups.Signals(12).XData = [0 10]
      | sbobj.Groups.Signals(12).YData = [1 1]
      | sbobj.Groups.Signals(13).Name = 'HealEnable'
      | sbobj.Groups.Signals(13).XData = [0 10]
      | sbobj.Groups.Signals(13).YData = [0 0]
      | sbobj.Groups.Signals(14).Name = 'PreestorageFreezeTrigger'
      | sbobj.Groups.Signals(14).XData = [0 10]
      | sbobj.Groups.Signals(14).YData = [1 1]
      | sbobj.Groups.Signals(15).Name = 'JumpDownEn'
      | sbobj.Groups.Signals(15).XData = [0 10]
      | sbobj.Groups.Signals(15).YData = [1 1]
  EnableSubsystem : Outport  Tag=STV Outport
  DiagInput : Outport  Tag=STV Outport  Port=2
  StartupComp : Outport  Tag=STV Outport  Port=3
  MaxValue : Outport  Tag=STV Outport  Port=4
  MinValue : Outport  Tag=STV Outport  Port=5
  UpCount : Outport  Tag=STV Outport  Port=6
  DownCount : Outport  Tag=STV Outport  Port=7
  FaultCountThd : Outport  Tag=STV Outport  Port=8
  PassCountThd : Outport  Tag=STV Outport  Port=9
  DebounceEn : Outport  Tag=STV Outport  Port=10
  DiagReset : Outport  Tag=STV Outport  Port=11
  DiagEnable : Outport  Tag=STV Outport  Port=12
  HealEnable : Outport  Tag=STV Outport  Port=13
  PreestorageFreezeTrigger : Outport  Tag=STV Outport  Port=14
  JumpDownEn : Outport  Tag=STV Outport  Port=15
  wires:
  Demux/15 -> JumpDownEn/1
  Demux/14 -> PreestorageFreezeTrigger/1
  Demux/13 -> HealEnable/1
  Demux/12 -> DiagEnable/1
  Demux/11 -> DiagReset/1
  Demux/10 -> DebounceEn/1
  Demux/9 -> PassCountThd/1
  Demux/8 -> FaultCountThd/1
  Demux/7 -> DownCount/1
  Demux/6 -> UpCount/1
  Demux/5 -> MinValue/1
  Demux/4 -> MaxValue/1
  Demux/3 -> StartupComp/1
  Demux/2 -> DiagInput/1
  Demux/1 -> EnableSubsystem/1
  FromWs/1 -> Demux/1

== system DiagCCaller_TestHarness/Debounce Enabled - RESET by Calibration ,Fault Active, FaultCnt = 10, PassCnt = -5, Heal 1 1/Signal Builder ==
  Demux : Demux  Tag=STV Demux  Outputs=15
  FromWs : FromWorkspace  Tag=STV FromWs  VariableName=tuvar  SampleTime=0
      SigBuilderData=|
      | common.afterFinalStr = 'Extrapolate'
      | common.sampleTime = 0
      | dataSet.timeRange = [0 10]
      | dataSet.name = 'Group 1'
      | sbobj.Groups.Name = 'Group 1'
      | sbobj.Groups.Signals(1).Name = 'EnableSubsystem'
      | sbobj.Groups.Signals(1).XData = [0 4.01 4.94 9.06 9.06 10]
      | sbobj.Groups.Signals(1).YData = [1 1 1 1 0 0]
      | sbobj.Groups.Signals(2).Name = 'DiagInput'
      | sbobj.Groups.Signals(2).XData = [0 2.5 4.17 6 6 7.51 7.51 8.99 8.99 10]
      | sbobj.Groups.Signals(2).YData = [1 1 1 1 0 0 1 1 0 0]
      | sbobj.Groups.Signals(3).Name = 'StartupComp'
      | sbobj.Groups.Signals(3).XData = [0 10]
      | sbobj.Groups.Signals(3).YData = [1 1]
      | sbobj.Groups.Signals(4).Name = 'MaxValue'
      | sbobj.Groups.Signals(4).XData = [0 10]
      | sbobj.Groups.Signals(4).YData = [9999 9999]
      | sbobj.Groups.Signals(5).Name = 'MinValue'
      | sbobj.Groups.Signals(5).XData = [0 10]
      | sbobj.Groups.Signals(5).YData = [-69.9 -69.9]
      | sbobj.Groups.Signals(6).Name = 'UpCount'
      | sbobj.Groups.Signals(6).XData = [0 10]
      | sbobj.Groups.Signals(6).YData = [1 1]
      | sbobj.Groups.Signals(7).Name = 'DownCount'
      | sbobj.Groups.Signals(7).XData = [0 10]
      | sbobj.Groups.Signals(7).YData = [1 1]
      | sbobj.Groups.Signals(8).Name = 'FaultCountThd'
      | sbobj.Groups.Signals(8).XData = [0 10]
      | sbobj.Groups.Signals(8).YData = [10 10]
      | sbobj.Groups.Signals(9).Name = 'PassCountThd'
      | sbobj.Groups.Signals(9).XData = [0 10]
      | sbobj.Groups.Signals(9).YData = [-5 -5]
      | sbobj.Groups.Signals(10).Name = 'DebounceEn'
      | sbobj.Groups.Signals(10).XData = [0 10]
      | sbobj.Groups.Signals(10).YData = [1 1]
      | sbobj.Groups.Signals(11).Name = 'DiagReset'
      | sbobj.Groups.Signals(11).XData = [0 3 3 4.73 4.73 10]
      | sbobj.Groups.Signals(11).YData = [0 0 1 1 0 0]
      | sbobj.Groups.Signals(12).Name = 'DiagEnable'
      | sbobj.Groups.Signals(12).XData = [0 10]
      | sbobj.Groups.Signals(12).YData = [1 1]
      | sbobj.Groups.Signals(13).Name = 'HealEnable'
      | sbobj.Groups.Signals(13).XData = [0 10]
      | sbobj.Groups.Signals(13).YData = [1 1]
      | sbobj.Groups.Signals(14).Name = 'PreestorageFreezeTrigger'
      | sbobj.Groups.Signals(14).XData = [0 10]
      | sbobj.Groups.Signals(14).YData = [1 1]
      | sbobj.Groups.Signals(15).Name = 'JumpDownEn'
      | sbobj.Groups.Signals(15).XData = [0 10]
      | sbobj.Groups.Signals(15).YData = [0 0]
  EnableSubsystem : Outport  Tag=STV Outport
  DiagInput : Outport  Tag=STV Outport  Port=2
  StartupComp : Outport  Tag=STV Outport  Port=3
  MaxValue : Outport  Tag=STV Outport  Port=4
  MinValue : Outport  Tag=STV Outport  Port=5
  UpCount : Outport  Tag=STV Outport  Port=6
  DownCount : Outport  Tag=STV Outport  Port=7
  FaultCountThd : Outport  Tag=STV Outport  Port=8
  PassCountThd : Outport  Tag=STV Outport  Port=9
  DebounceEn : Outport  Tag=STV Outport  Port=10
  DiagReset : Outport  Tag=STV Outport  Port=11
  DiagEnable : Outport  Tag=STV Outport  Port=12
  HealEnable : Outport  Tag=STV Outport  Port=13
  PreestorageFreezeTrigger : Outport  Tag=STV Outport  Port=14
  JumpDownEn : Outport  Tag=STV Outport  Port=15
  wires:
  FromWs/1 -> Demux/1
  Demux/1 -> EnableSubsystem/1
  Demux/2 -> DiagInput/1
  Demux/3 -> StartupComp/1
  Demux/4 -> MaxValue/1
  Demux/5 -> MinValue/1
  Demux/6 -> UpCount/1
  Demux/7 -> DownCount/1
  Demux/8 -> FaultCountThd/1
  Demux/9 -> PassCountThd/1
  Demux/10 -> DebounceEn/1
  Demux/11 -> DiagReset/1
  Demux/12 -> DiagEnable/1
  Demux/13 -> HealEnable/1
  Demux/14 -> PreestorageFreezeTrigger/1
  Demux/15 -> JumpDownEn/1

== system DiagCCaller_TestHarness/Debounce Enabled - RESET by Calibration ,Fault Active, FaultCnt = 10, PassCnt = 0 , Heal 0 /Signal Builder ==
  Demux : Demux  Tag=STV Demux  Outputs=15
  FromWs : FromWorkspace  Tag=STV FromWs  VariableName=tuvar  SampleTime=0
      SigBuilderData=|
      | common.afterFinalStr = 'Extrapolate'
      | common.sampleTime = 0
      | dataSet.timeRange = [0 10]
      | dataSet.name = 'Group 1'
      | sbobj.Groups.Name = 'Group 1'
      | sbobj.Groups.Signals(1).Name = 'EnableSubsystem'
      | sbobj.Groups.Signals(1).XData = [0 4.01 4.94 9.06 9.06 10]
      | sbobj.Groups.Signals(1).YData = [1 1 1 1 0 0]
      | sbobj.Groups.Signals(2).Name = 'DiagInput'
      | sbobj.Groups.Signals(2).XData = [0 2.5 4.17 6 6 7.51 7.51 8.99 8.99 10]
      | sbobj.Groups.Signals(2).YData = [1 1 1 1 0 0 1 1 0 0]
      | sbobj.Groups.Signals(3).Name = 'StartupComp'
      | sbobj.Groups.Signals(3).XData = [0 10]
      | sbobj.Groups.Signals(3).YData = [1 1]
      | sbobj.Groups.Signals(4).Name = 'MaxValue'
      | sbobj.Groups.Signals(4).XData = [0 10]
      | sbobj.Groups.Signals(4).YData = [9999 9999]
      | sbobj.Groups.Signals(5).Name = 'MinValue'
      | sbobj.Groups.Signals(5).XData = [0 10]
      | sbobj.Groups.Signals(5).YData = [-69.9 -69.9]
      | sbobj.Groups.Signals(6).Name = 'UpCount'
      | sbobj.Groups.Signals(6).XData = [0 10]
      | sbobj.Groups.Signals(6).YData = [1 1]
      | sbobj.Groups.Signals(7).Name = 'DownCount'
      | sbobj.Groups.Signals(7).XData = [0 10]
      | sbobj.Groups.Signals(7).YData = [1 1]
      | sbobj.Groups.Signals(8).Name = 'FaultCountThd'
      | sbobj.Groups.Signals(8).XData = [0 10]
      | sbobj.Groups.Signals(8).YData = [10 10]
      | sbobj.Groups.Signals(9).Name = 'PassCountThd'
      | sbobj.Groups.Signals(9).XData = [0 10]
      | sbobj.Groups.Signals(9).YData = [0 0]
      | sbobj.Groups.Signals(10).Name = 'DebounceEn'
      | sbobj.Groups.Signals(10).XData = [0 10]
      | sbobj.Groups.Signals(10).YData = [1 1]
      | sbobj.Groups.Signals(11).Name = 'DiagReset'
      | sbobj.Groups.Signals(11).XData = [0 3 3 4.73 4.73 10]
      | sbobj.Groups.Signals(11).YData = [0 0 1 1 0 0]
      | sbobj.Groups.Signals(12).Name = 'DiagEnable'
      | sbobj.Groups.Signals(12).XData = [0 10]
      | sbobj.Groups.Signals(12).YData = [1 1]
      | sbobj.Groups.Signals(13).Name = 'HealEnable'
      | sbobj.Groups.Signals(13).XData = [0 10]
      | sbobj.Groups.Signals(13).YData = [0 0]
      | sbobj.Groups.Signals(14).Name = 'PreestorageFreezeTrigger'
      | sbobj.Groups.Signals(14).XData = [0 10]
      | sbobj.Groups.Signals(14).YData = [1 1]
      | sbobj.Groups.Signals(15).Name = 'JumpDownEn'
      | sbobj.Groups.Signals(15).XData = [0 10]
      | sbobj.Groups.Signals(15).YData = [1 1]
  EnableSubsystem : Outport  Tag=STV Outport
  DiagInput : Outport  Tag=STV Outport  Port=2
  StartupComp : Outport  Tag=STV Outport  Port=3
  MaxValue : Outport  Tag=STV Outport  Port=4
  MinValue : Outport  Tag=STV Outport  Port=5
  UpCount : Outport  Tag=STV Outport  Port=6
  DownCount : Outport  Tag=STV Outport  Port=7
  FaultCountThd : Outport  Tag=STV Outport  Port=8
  PassCountThd : Outport  Tag=STV Outport  Port=9
  DebounceEn : Outport  Tag=STV Outport  Port=10
  DiagReset : Outport  Tag=STV Outport  Port=11
  DiagEnable : Outport  Tag=STV Outport  Port=12
  HealEnable : Outport  Tag=STV Outport  Port=13
  PreestorageFreezeTrigger : Outport  Tag=STV Outport  Port=14
  JumpDownEn : Outport  Tag=STV Outport  Port=15
  wires:
  FromWs/1 -> Demux/1
  Demux/1 -> EnableSubsystem/1
  Demux/2 -> DiagInput/1
  Demux/3 -> StartupComp/1
  Demux/4 -> MaxValue/1
  Demux/5 -> MinValue/1
  Demux/6 -> UpCount/1
  Demux/7 -> DownCount/1
  Demux/8 -> FaultCountThd/1
  Demux/9 -> PassCountThd/1
  Demux/10 -> DebounceEn/1
  Demux/11 -> DiagReset/1
  Demux/12 -> DiagEnable/1
  Demux/13 -> HealEnable/1
  Demux/14 -> PreestorageFreezeTrigger/1
  Demux/15 -> JumpDownEn/1

== system DiagCCaller_TestHarness/Debounce Enabled - RESET by Calibration ,Fault Inactive , FaultCnt = 10, PassCnt = 0 , Heal 0 /Signal Builder ==
  Demux : Demux  Tag=STV Demux  Outputs=15
  FromWs : FromWorkspace  Tag=STV FromWs  VariableName=tuvar  SampleTime=0
      SigBuilderData=|
      | common.afterFinalStr = 'Extrapolate'
      | common.sampleTime = 0
      | dataSet.timeRange = [0 10]
      | dataSet.name = 'Group 1'
      | sbobj.Groups.Name = 'Group 1'
      | sbobj.Groups.Signals(1).Name = 'EnableSubsystem'
      | sbobj.Groups.Signals(1).XData = [0 4.36 4.94 9.06 9.06 10]
      | sbobj.Groups.Signals(1).YData = [1 1 1 1 0 0]
      | sbobj.Groups.Signals(2).Name = 'DiagInput'
      | sbobj.Groups.Signals(2).XData = [0 1 3.94 3.94 6 6 8 8 9.5 9.5 10]
      | sbobj.Groups.Signals(2).YData = [0 0 0 1.1 1.1 0 0 1.2 1.2 0 0]
      | sbobj.Groups.Signals(3).Name = 'StartupComp'
      | sbobj.Groups.Signals(3).XData = [0 10]
      | sbobj.Groups.Signals(3).YData = [1 1]
      | sbobj.Groups.Signals(4).Name = 'MaxValue'
      | sbobj.Groups.Signals(4).XData = [0 10]
      | sbobj.Groups.Signals(4).YData = [9999 9999]
      | sbobj.Groups.Signals(5).Name = 'MinValue'
      | sbobj.Groups.Signals(5).XData = [0 10]
      | sbobj.Groups.Signals(5).YData = [-69.9 -69.9]
      | sbobj.Groups.Signals(6).Name = 'UpCount'
      | sbobj.Groups.Signals(6).XData = [0 10]
      | sbobj.Groups.Signals(6).YData = [1 1]
      | sbobj.Groups.Signals(7).Name = 'DownCount'
      | sbobj.Groups.Signals(7).XData = [0 10]
      | sbobj.Groups.Signals(7).YData = [1 1]
      | sbobj.Groups.Signals(8).Name = 'FaultCountThd'
      | sbobj.Groups.Signals(8).XData = [0 10]
      | sbobj.Groups.Signals(8).YData = [10 10]
      | sbobj.Groups.Signals(9).Name = 'PassCountThd'
      | sbobj.Groups.Signals(9).XData = [0 10]
      | sbobj.Groups.Signals(9).YData = [0 0]
      | sbobj.Groups.Signals(10).Name = 'DebounceEn'
      | sbobj.Groups.Signals(10).XData = [0 10]
      | sbobj.Groups.Signals(10).YData = [1 1]
      | sbobj.Groups.Signals(11).Name = 'DiagReset'
      | sbobj.Groups.Signals(11).XData = [0 1.33 1.33 2.66 2.66 10]
      | sbobj.Groups.Signals(11).YData = [0 0 1 1 0 0]
      | sbobj.Groups.Signals(12).Name = 'DiagEnable'
      | sbobj.Groups.Signals(12).XData = [0 10]
      | sbobj.Groups.Signals(12).YData = [1 1]
      | sbobj.Groups.Signals(13).Name = 'HealEnable'
      | sbobj.Groups.Signals(13).XData = [0 10]
      | sbobj.Groups.Signals(13).YData = [0 0]
      | sbobj.Groups.Signals(14).Name = 'PreestorageFreezeTrigger'
      | sbobj.Groups.Signals(14).XData = [0 10]
      | sbobj.Groups.Signals(14).YData = [1 1]
      | sbobj.Groups.Signals(15).Name = 'JumpDownEn'
      | sbobj.Groups.Signals(15).XData = [0 10]
      | sbobj.Groups.Signals(15).YData = [1 1]
  EnableSubsystem : Outport  Tag=STV Outport
  DiagInput : Outport  Tag=STV Outport  Port=2
  StartupComp : Outport  Tag=STV Outport  Port=3
  MaxValue : Outport  Tag=STV Outport  Port=4
  MinValue : Outport  Tag=STV Outport  Port=5
  UpCount : Outport  Tag=STV Outport  Port=6
  DownCount : Outport  Tag=STV Outport  Port=7
  FaultCountThd : Outport  Tag=STV Outport  Port=8
  PassCountThd : Outport  Tag=STV Outport  Port=9
  DebounceEn : Outport  Tag=STV Outport  Port=10
  DiagReset : Outport  Tag=STV Outport  Port=11
  DiagEnable : Outport  Tag=STV Outport  Port=12
  HealEnable : Outport  Tag=STV Outport  Port=13
  PreestorageFreezeTrigger : Outport  Tag=STV Outport  Port=14
  JumpDownEn : Outport  Tag=STV Outport  Port=15
  wires:
  Demux/15 -> JumpDownEn/1
  Demux/14 -> PreestorageFreezeTrigger/1
  Demux/13 -> HealEnable/1
  Demux/12 -> DiagEnable/1
  Demux/11 -> DiagReset/1
  Demux/10 -> DebounceEn/1
  Demux/9 -> PassCountThd/1
  Demux/8 -> FaultCountThd/1
  Demux/7 -> DownCount/1
  Demux/6 -> UpCount/1
  Demux/5 -> MinValue/1
  Demux/4 -> MaxValue/1
  Demux/3 -> StartupComp/1
  Demux/2 -> DiagInput/1
  Demux/1 -> EnableSubsystem/1
  FromWs/1 -> Demux/1

== system DiagCCaller_TestHarness/Debounce Enabled - RESET by Calibration ,Fault Inactive,  FaultCnt = 10, PassCnt = -5 , Heal 1 /Signal Builder ==
  Demux : Demux  Tag=STV Demux  Outputs=15
  FromWs : FromWorkspace  Tag=STV FromWs  VariableName=tuvar  SampleTime=0
      SigBuilderData=|
      | common.afterFinalStr = 'Extrapolate'
      | common.sampleTime = 0
      | dataSet.timeRange = [0 10]
      | dataSet.name = 'Group 1'
      | sbobj.Groups.Name = 'Group 1'
      | sbobj.Groups.Signals(1).Name = 'EnableSubsystem'
      | sbobj.Groups.Signals(1).XData = [0 4.36 4.94 9.06 9.06 10]
      | sbobj.Groups.Signals(1).YData = [1 1 1 1 0 0]
      | sbobj.Groups.Signals(2).Name = 'DiagInput'
      | sbobj.Groups.Signals(2).XData = [0 1 2.41 3.88 3.88 6 6 8 8 9.5 9.5 10]
      | sbobj.Groups.Signals(2).YData = [0 0 0 0 1.1 1.1 0 0 1.2 1.2 0 0]
      | sbobj.Groups.Signals(3).Name = 'StartupComp'
      | sbobj.Groups.Signals(3).XData = [0 10]
      | sbobj.Groups.Signals(3).YData = [1 1]
      | sbobj.Groups.Signals(4).Name = 'MaxValue'
      | sbobj.Groups.Signals(4).XData = [0 10]
      | sbobj.Groups.Signals(4).YData = [9999 9999]
      | sbobj.Groups.Signals(5).Name = 'MinValue'
      | sbobj.Groups.Signals(5).XData = [0 10]
      | sbobj.Groups.Signals(5).YData = [-69.9 -69.9]
      | sbobj.Groups.Signals(6).Name = 'UpCount'
      | sbobj.Groups.Signals(6).XData = [0 10]
      | sbobj.Groups.Signals(6).YData = [1 1]
      | sbobj.Groups.Signals(7).Name = 'DownCount'
      | sbobj.Groups.Signals(7).XData = [0 10]
      | sbobj.Groups.Signals(7).YData = [1 1]
      | sbobj.Groups.Signals(8).Name = 'FaultCountThd'
      | sbobj.Groups.Signals(8).XData = [0 10]
      | sbobj.Groups.Signals(8).YData = [10 10]
      | sbobj.Groups.Signals(9).Name = 'PassCountThd'
      | sbobj.Groups.Signals(9).XData = [0 10]
      | sbobj.Groups.Signals(9).YData = [-5 -5]
      | sbobj.Groups.Signals(10).Name = 'DebounceEn'
      | sbobj.Groups.Signals(10).XData = [0 10]
      | sbobj.Groups.Signals(10).YData = [1 1]
      | sbobj.Groups.Signals(11).Name = 'DiagReset'
      | sbobj.Groups.Signals(11).XData = [0 1.74 1.74 2.79 2.79 10]
      | sbobj.Groups.Signals(11).YData = [0 0 1 1 0 0]
      | sbobj.Groups.Signals(12).Name = 'DiagEnable'
      | sbobj.Groups.Signals(12).XData = [0 10]
      | sbobj.Groups.Signals(12).YData = [1 1]
      | sbobj.Groups.Signals(13).Name = 'HealEnable'
      | sbobj.Groups.Signals(13).XData = [0 10]
      | sbobj.Groups.Signals(13).YData = [1 1]
      | sbobj.Groups.Signals(14).Name = 'PreestorageFreezeTrigger'
      | sbobj.Groups.Signals(14).XData = [0 10]
      | sbobj.Groups.Signals(14).YData = [1 1]
      | sbobj.Groups.Signals(15).Name = 'JumpDownEn'
      | sbobj.Groups.Signals(15).XData = [0 10]
      | sbobj.Groups.Signals(15).YData = [0 0]
  EnableSubsystem : Outport  Tag=STV Outport
  DiagInput : Outport  Tag=STV Outport  Port=2
  StartupComp : Outport  Tag=STV Outport  Port=3
  MaxValue : Outport  Tag=STV Outport  Port=4
  MinValue : Outport  Tag=STV Outport  Port=5
  UpCount : Outport  Tag=STV Outport  Port=6
  DownCount : Outport  Tag=STV Outport  Port=7
  FaultCountThd : Outport  Tag=STV Outport  Port=8
  PassCountThd : Outport  Tag=STV Outport  Port=9
  DebounceEn : Outport  Tag=STV Outport  Port=10
  DiagReset : Outport  Tag=STV Outport  Port=11
  DiagEnable : Outport  Tag=STV Outport  Port=12
  HealEnable : Outport  Tag=STV Outport  Port=13
  PreestorageFreezeTrigger : Outport  Tag=STV Outport  Port=14
  JumpDownEn : Outport  Tag=STV Outport  Port=15
  wires:
  FromWs/1 -> Demux/1
  Demux/1 -> EnableSubsystem/1
  Demux/2 -> DiagInput/1
  Demux/3 -> StartupComp/1
  Demux/4 -> MaxValue/1
  Demux/5 -> MinValue/1
  Demux/6 -> UpCount/1
  Demux/7 -> DownCount/1
  Demux/8 -> FaultCountThd/1
  Demux/9 -> PassCountThd/1
  Demux/10 -> DebounceEn/1
  Demux/11 -> DiagReset/1
  Demux/12 -> DiagEnable/1
  Demux/13 -> HealEnable/1
  Demux/14 -> PreestorageFreezeTrigger/1
  Demux/15 -> JumpDownEn/1

== system DiagCCaller_TestHarness/Debounce Enabled - RESET by Disable\Enable subsystem,Fault Active, FaultCnt = 10, PassCnt = -5, Heal 1 /Signal Builder ==
  Demux : Demux  Tag=STV Demux  Outputs=15
  FromWs : FromWorkspace  Tag=STV FromWs  VariableName=tuvar  SampleTime=0
      SigBuilderData=|
      | common.afterFinalStr = 'Extrapolate'
      | common.sampleTime = 0
      | dataSet.timeRange = [0 10]
      | dataSet.name = 'Group 1'
      | sbobj.Groups.Name = 'Group 1'
      | sbobj.Groups.Signals(1).Name = 'EnableSubsystem'
      | sbobj.Groups.Signals(1).XData = [0 3.58 3.58 5.02 5.02 7.23 7.23 8.06 8.06 9.06 9.06 10]
      | sbobj.Groups.Signals(1).YData = [1 1 0 0 1 1 0 0 1 1 0 0]
      | sbobj.Groups.Signals(2).Name = 'DiagInput'
      | sbobj.Groups.Signals(2).XData = [0 1 2.41 2.41 6.22 6.22 8 8 9.5 9.5 10]
      | sbobj.Groups.Signals(2).YData = [0 0 0 1.1 1.1 0 0 1.2 1.2 0 0]
      | sbobj.Groups.Signals(3).Name = 'StartupComp'
      | sbobj.Groups.Signals(3).XData = [0 10]
      | sbobj.Groups.Signals(3).YData = [1 1]
      | sbobj.Groups.Signals(4).Name = 'MaxValue'
      | sbobj.Groups.Signals(4).XData = [0 10]
      | sbobj.Groups.Signals(4).YData = [9999 9999]
      | sbobj.Groups.Signals(5).Name = 'MinValue'
      | sbobj.Groups.Signals(5).XData = [0 10]
      | sbobj.Groups.Signals(5).YData = [-69.9 -69.9]
      | sbobj.Groups.Signals(6).Name = 'UpCount'
      | sbobj.Groups.Signals(6).XData = [0 10]
      | sbobj.Groups.Signals(6).YData = [1 1]
      | sbobj.Groups.Signals(7).Name = 'DownCount'
      | sbobj.Groups.Signals(7).XData = [0 10]
      | sbobj.Groups.Signals(7).YData = [1 1]
      | sbobj.Groups.Signals(8).Name = 'FaultCountThd'
      | sbobj.Groups.Signals(8).XData = [0 10]
      | sbobj.Groups.Signals(8).YData = [10 10]
      | sbobj.Groups.Signals(9).Name = 'PassCountThd'
      | sbobj.Groups.Signals(9).XData = [0 10]
      | sbobj.Groups.Signals(9).YData = [-5 -5]
      | sbobj.Groups.Signals(10).Name = 'DebounceEn'
      | sbobj.Groups.Signals(10).XData = [0 10]
      | sbobj.Groups.Signals(10).YData = [1 1]
      | sbobj.Groups.Signals(11).Name = 'DiagReset'
      | sbobj.Groups.Signals(11).XData = [0 5.34 5.34 6.12 6.12 7.7 10]
      | sbobj.Groups.Signals(11).YData = [0 0 1 1 0 0 0]
      | sbobj.Groups.Signals(12).Name = 'DiagEnable'
      | sbobj.Groups.Signals(12).XData = [0 10]
      | sbobj.Groups.Signals(12).YData = [1 1]
      | sbobj.Groups.Signals(13).Name = 'HealEnable'
      | sbobj.Groups.Signals(13).XData = [0 10]
      | sbobj.Groups.Signals(13).YData = [1 1]
      | sbobj.Groups.Signals(14).Name = 'PreestorageFreezeTrigger'
      | sbobj.Groups.Signals(14).XData = [0 10]
      | sbobj.Groups.Signals(14).YData = [1 1]
      | sbobj.Groups.Signals(15).Name = 'JumpDownEn'
      | sbobj.Groups.Signals(15).XData = [0 10]
      | sbobj.Groups.Signals(15).YData = [0 0]
  EnableSubsystem : Outport  Tag=STV Outport
  DiagInput : Outport  Tag=STV Outport  Port=2
  StartupComp : Outport  Tag=STV Outport  Port=3
  MaxValue : Outport  Tag=STV Outport  Port=4
  MinValue : Outport  Tag=STV Outport  Port=5
  UpCount : Outport  Tag=STV Outport  Port=6
  DownCount : Outport  Tag=STV Outport  Port=7
  FaultCountThd : Outport  Tag=STV Outport  Port=8
  PassCountThd : Outport  Tag=STV Outport  Port=9
  DebounceEn : Outport  Tag=STV Outport  Port=10
  DiagReset : Outport  Tag=STV Outport  Port=11
  DiagEnable : Outport  Tag=STV Outport  Port=12
  HealEnable : Outport  Tag=STV Outport  Port=13
  PreestorageFreezeTrigger : Outport  Tag=STV Outport  Port=14
  JumpDownEn : Outport  Tag=STV Outport  Port=15
  wires:
  FromWs/1 -> Demux/1
  Demux/1 -> EnableSubsystem/1
  Demux/2 -> DiagInput/1
  Demux/3 -> StartupComp/1
  Demux/4 -> MaxValue/1
  Demux/5 -> MinValue/1
  Demux/6 -> UpCount/1
  Demux/7 -> DownCount/1
  Demux/8 -> FaultCountThd/1
  Demux/9 -> PassCountThd/1
  Demux/10 -> DebounceEn/1
  Demux/11 -> DiagReset/1
  Demux/12 -> DiagEnable/1
  Demux/13 -> HealEnable/1
  Demux/14 -> PreestorageFreezeTrigger/1
  Demux/15 -> JumpDownEn/1

== system DiagCCaller_TestHarness/Debounce Enabled - RESET by Disable\Enable subsystem,Fault Active, FaultCnt = 10, PassCnt = 0 , Heal 0 /Signal Builder ==
  Demux : Demux  Tag=STV Demux  Outputs=15
  FromWs : FromWorkspace  Tag=STV FromWs  VariableName=tuvar  SampleTime=0
      SigBuilderData=|
      | common.afterFinalStr = 'Extrapolate'
      | common.sampleTime = 0
      | dataSet.timeRange = [0 10]
      | dataSet.name = 'Group 1'
      | sbobj.Groups.Name = 'Group 1'
      | sbobj.Groups.Signals(1).Name = 'EnableSubsystem'
      | sbobj.Groups.Signals(1).XData = [0 4.36 4.36 4.94 4.94 9.06 9.06 10]
      | sbobj.Groups.Signals(1).YData = [1 1 0 0 1 1 0 0]
      | sbobj.Groups.Signals(2).Name = 'DiagInput'
      | sbobj.Groups.Signals(2).XData = [0 1 2.5 2.5 7.04 7.04 7.04 8 8 9.5 9.5 10]
      | sbobj.Groups.Signals(2).YData = [0 0 0 1 1 0 0 0 1.2 1.2 0 0]
      | sbobj.Groups.Signals(3).Name = 'StartupComp'
      | sbobj.Groups.Signals(3).XData = [0 10]
      | sbobj.Groups.Signals(3).YData = [1 1]
      | sbobj.Groups.Signals(4).Name = 'MaxValue'
      | sbobj.Groups.Signals(4).XData = [0 10]
      | sbobj.Groups.Signals(4).YData = [9999 9999]
      | sbobj.Groups.Signals(5).Name = 'MinValue'
      | sbobj.Groups.Signals(5).XData = [0 10]
      | sbobj.Groups.Signals(5).YData = [-69.9 -69.9]
      | sbobj.Groups.Signals(6).Name = 'UpCount'
      | sbobj.Groups.Signals(6).XData = [0 10]
      | sbobj.Groups.Signals(6).YData = [1 1]
      | sbobj.Groups.Signals(7).Name = 'DownCount'
      | sbobj.Groups.Signals(7).XData = [0 10]
      | sbobj.Groups.Signals(7).YData = [1 1]
      | sbobj.Groups.Signals(8).Name = 'FaultCountThd'
      | sbobj.Groups.Signals(8).XData = [0 10]
      | sbobj.Groups.Signals(8).YData = [10 10]
      | sbobj.Groups.Signals(9).Name = 'PassCountThd'
      | sbobj.Groups.Signals(9).XData = [0 10]
      | sbobj.Groups.Signals(9).YData = [0 0]
      | sbobj.Groups.Signals(10).Name = 'DebounceEn'
      | sbobj.Groups.Signals(10).XData = [0 10]
      | sbobj.Groups.Signals(10).YData = [1 1]
      | sbobj.Groups.Signals(11).Name = 'DiagReset'
      | sbobj.Groups.Signals(11).XData = [0 10]
      | sbobj.Groups.Signals(11).YData = [0 0]
      | sbobj.Groups.Signals(12).Name = 'DiagEnable'
      | sbobj.Groups.Signals(12).XData = [0 10]
      | sbobj.Groups.Signals(12).YData = [1 1]
      | sbobj.Groups.Signals(13).Name = 'HealEnable'
      | sbobj.Groups.Signals(13).XData = [0 10]
      | sbobj.Groups.Signals(13).YData = [0 0]
      | sbobj.Groups.Signals(14).Name = 'PreestorageFreezeTrigger'
      | sbobj.Groups.Signals(14).XData = [0 10]
      | sbobj.Groups.Signals(14).YData = [1 1]
      | sbobj.Groups.Signals(15).Name = 'JumpDownEn'
      | sbobj.Groups.Signals(15).XData = [0 10]
      | sbobj.Groups.Signals(15).YData = [1 1]
  EnableSubsystem : Outport  Tag=STV Outport
  DiagInput : Outport  Tag=STV Outport  Port=2
  StartupComp : Outport  Tag=STV Outport  Port=3
  MaxValue : Outport  Tag=STV Outport  Port=4
  MinValue : Outport  Tag=STV Outport  Port=5
  UpCount : Outport  Tag=STV Outport  Port=6
  DownCount : Outport  Tag=STV Outport  Port=7
  FaultCountThd : Outport  Tag=STV Outport  Port=8
  PassCountThd : Outport  Tag=STV Outport  Port=9
  DebounceEn : Outport  Tag=STV Outport  Port=10
  DiagReset : Outport  Tag=STV Outport  Port=11
  DiagEnable : Outport  Tag=STV Outport  Port=12
  HealEnable : Outport  Tag=STV Outport  Port=13
  PreestorageFreezeTrigger : Outport  Tag=STV Outport  Port=14
  JumpDownEn : Outport  Tag=STV Outport  Port=15
  wires:
  Demux/15 -> JumpDownEn/1
  Demux/14 -> PreestorageFreezeTrigger/1
  Demux/13 -> HealEnable/1
  Demux/12 -> DiagEnable/1
  Demux/11 -> DiagReset/1
  Demux/10 -> DebounceEn/1
  Demux/9 -> PassCountThd/1
  Demux/8 -> FaultCountThd/1
  Demux/7 -> DownCount/1
  Demux/6 -> UpCount/1
  Demux/5 -> MinValue/1
  Demux/4 -> MaxValue/1
  Demux/3 -> StartupComp/1
  Demux/2 -> DiagInput/1
  Demux/1 -> EnableSubsystem/1
  FromWs/1 -> Demux/1

== system DiagCCaller_TestHarness/Debounce Enabled - RESET by Disable\Enable subsystem,Fault Inactive,  FaultCnt = 10, PassCnt = -5 , Heal 1 /Signal Builder ==
  Demux : Demux  Tag=STV Demux  Outputs=15
  FromWs : FromWorkspace  Tag=STV FromWs  VariableName=tuvar  SampleTime=0
      SigBuilderData=|
      | common.afterFinalStr = 'Extrapolate'
      | common.sampleTime = 0
      | dataSet.timeRange = [0 10]
      | dataSet.name = 'Group 1'
      | sbobj.Groups.Name = 'Group 1'
      | sbobj.Groups.Signals(1).Name = 'EnableSubsystem'
      | sbobj.Groups.Signals(1).XData = [0 1.99 1.99 2.98 2.98 4.36 4.94 9.06 9.06 10]
      | sbobj.Groups.Signals(1).YData = [1 1 0 0 1 1 1 1 0 0]
      | sbobj.Groups.Signals(2).Name = 'DiagInput'
      | sbobj.Groups.Signals(2).XData = [0 1.7 2.41 4.58 4.58 6 6 8 8 9.5 9.5 10]
      | sbobj.Groups.Signals(2).YData = [0 0 0 0 1.1 1.1 0 0 1.2 1.2 0 0]
      | sbobj.Groups.Signals(3).Name = 'StartupComp'
      | sbobj.Groups.Signals(3).XData = [0 10]
      | sbobj.Groups.Signals(3).YData = [1 1]
      | sbobj.Groups.Signals(4).Name = 'MaxValue'
      | sbobj.Groups.Signals(4).XData = [0 10]
      | sbobj.Groups.Signals(4).YData = [9999 9999]
      | sbobj.Groups.Signals(5).Name = 'MinValue'
      | sbobj.Groups.Signals(5).XData = [0 10]
      | sbobj.Groups.Signals(5).YData = [-69.9 -69.9]
      | sbobj.Groups.Signals(6).Name = 'UpCount'
      | sbobj.Groups.Signals(6).XData = [0 10]
      | sbobj.Groups.Signals(6).YData = [1 1]
      | sbobj.Groups.Signals(7).Name = 'DownCount'
      | sbobj.Groups.Signals(7).XData = [0 10]
      | sbobj.Groups.Signals(7).YData = [1 1]
      | sbobj.Groups.Signals(8).Name = 'FaultCountThd'
      | sbobj.Groups.Signals(8).XData = [0 10]
      | sbobj.Groups.Signals(8).YData = [10 10]
      | sbobj.Groups.Signals(9).Name = 'PassCountThd'
      | sbobj.Groups.Signals(9).XData = [0 10]
      | sbobj.Groups.Signals(9).YData = [-5 -5]
      | sbobj.Groups.Signals(10).Name = 'DebounceEn'
      | sbobj.Groups.Signals(10).XData = [0 10]
      | sbobj.Groups.Signals(10).YData = [1 1]
      | sbobj.Groups.Signals(11).Name = 'DiagReset'
      | sbobj.Groups.Signals(11).XData = [0 10]
      | sbobj.Groups.Signals(11).YData = [0 0]
      | sbobj.Groups.Signals(12).Name = 'DiagEnable'
      | sbobj.Groups.Signals(12).XData = [0 10]
      | sbobj.Groups.Signals(12).YData = [1 1]
      | sbobj.Groups.Signals(13).Name = 'HealEnable'
      | sbobj.Groups.Signals(13).XData = [0 10]
      | sbobj.Groups.Signals(13).YData = [1 1]
      | sbobj.Groups.Signals(14).Name = 'PreestorageFreezeTrigger'
      | sbobj.Groups.Signals(14).XData = [0 10]
      | sbobj.Groups.Signals(14).YData = [1 1]
      | sbobj.Groups.Signals(15).Name = 'JumpDownEn'
      | sbobj.Groups.Signals(15).XData = [0 10]
      | sbobj.Groups.Signals(15).YData = [0 0]
  EnableSubsystem : Outport  Tag=STV Outport
  DiagInput : Outport  Tag=STV Outport  Port=2
  StartupComp : Outport  Tag=STV Outport  Port=3
  MaxValue : Outport  Tag=STV Outport  Port=4
  MinValue : Outport  Tag=STV Outport  Port=5
  UpCount : Outport  Tag=STV Outport  Port=6
  DownCount : Outport  Tag=STV Outport  Port=7
  FaultCountThd : Outport  Tag=STV Outport  Port=8
  PassCountThd : Outport  Tag=STV Outport  Port=9
  DebounceEn : Outport  Tag=STV Outport  Port=10
  DiagReset : Outport  Tag=STV Outport  Port=11
  DiagEnable : Outport  Tag=STV Outport  Port=12
  HealEnable : Outport  Tag=STV Outport  Port=13
  PreestorageFreezeTrigger : Outport  Tag=STV Outport  Port=14
  JumpDownEn : Outport  Tag=STV Outport  Port=15
  wires:
  Demux/15 -> JumpDownEn/1
  Demux/14 -> PreestorageFreezeTrigger/1
  Demux/13 -> HealEnable/1
  Demux/12 -> DiagEnable/1
  Demux/11 -> DiagReset/1
  Demux/10 -> DebounceEn/1
  Demux/9 -> PassCountThd/1
  Demux/8 -> FaultCountThd/1
  Demux/7 -> DownCount/1
  Demux/6 -> UpCount/1
  Demux/5 -> MinValue/1
  Demux/4 -> MaxValue/1
  Demux/3 -> StartupComp/1
  Demux/2 -> DiagInput/1
  Demux/1 -> EnableSubsystem/1
  FromWs/1 -> Demux/1

== system DiagCCaller_TestHarness/Debounce Enabled - RESET by Disable\Enable subsystem,Fault Inactive, , FaultCnt = 10, PassCnt = 0 , Heal 0 /Signal Builder ==
  Demux : Demux  Tag=STV Demux  Outputs=15
  FromWs : FromWorkspace  Tag=STV FromWs  VariableName=tuvar  SampleTime=0
      SigBuilderData=|
      | common.afterFinalStr = 'Extrapolate'
      | common.sampleTime = 0
      | dataSet.timeRange = [0 10]
      | dataSet.name = 'Group 1'
      | sbobj.Groups.Name = 'Group 1'
      | sbobj.Groups.Signals(1).Name = 'EnableSubsystem'
      | sbobj.Groups.Signals(1).XData = [0 2.59 2.59 3.42 3.42 4.36 4.94 9.06 9.06 10]
      | sbobj.Groups.Signals(1).YData = [1 1 0 0 1 1 1 1 0 0]
      | sbobj.Groups.Signals(2).Name = 'DiagInput'
      | sbobj.Groups.Signals(2).XData = [0 1 2.41 4.96 4.96 7.09 7.09 8.36 8.36 9.5 9.5 10]
      | sbobj.Groups.Signals(2).YData = [0 0 0 0 1.1 1.1 0 0 1.2 1.2 0 0]
      | sbobj.Groups.Signals(3).Name = 'StartupComp'
      | sbobj.Groups.Signals(3).XData = [0 10]
      | sbobj.Groups.Signals(3).YData = [1 1]
      | sbobj.Groups.Signals(4).Name = 'MaxValue'
      | sbobj.Groups.Signals(4).XData = [0 10]
      | sbobj.Groups.Signals(4).YData = [9999 9999]
      | sbobj.Groups.Signals(5).Name = 'MinValue'
      | sbobj.Groups.Signals(5).XData = [0 10]
      | sbobj.Groups.Signals(5).YData = [-69.9 -69.9]
      | sbobj.Groups.Signals(6).Name = 'UpCount'
      | sbobj.Groups.Signals(6).XData = [0 10]
      | sbobj.Groups.Signals(6).YData = [1 1]
      | sbobj.Groups.Signals(7).Name = 'DownCount'
      | sbobj.Groups.Signals(7).XData = [0 10]
      | sbobj.Groups.Signals(7).YData = [1 1]
      | sbobj.Groups.Signals(8).Name = 'FaultCountThd'
      | sbobj.Groups.Signals(8).XData = [0 10]
      | sbobj.Groups.Signals(8).YData = [10 10]
      | sbobj.Groups.Signals(9).Name = 'PassCountThd'
      | sbobj.Groups.Signals(9).XData = [0 10]
      | sbobj.Groups.Signals(9).YData = [0 0]
      | sbobj.Groups.Signals(10).Name = 'DebounceEn'
      | sbobj.Groups.Signals(10).XData = [0 10]
      | sbobj.Groups.Signals(10).YData = [1 1]
      | sbobj.Groups.Signals(11).Name = 'DiagReset'
      | sbobj.Groups.Signals(11).XData = [0 10]
      | sbobj.Groups.Signals(11).YData = [0 0]
      | sbobj.Groups.Signals(12).Name = 'DiagEnable'
      | sbobj.Groups.Signals(12).XData = [0 5.37 5.37 6.72 6.72 10]
      | sbobj.Groups.Signals(12).YData = [1 1 0 0 1 1]
      | sbobj.Groups.Signals(13).Name = 'HealEnable'
      | sbobj.Groups.Signals(13).XData = [0 10]
      | sbobj.Groups.Signals(13).YData = [0 0]
      | sbobj.Groups.Signals(14).Name = 'PreestorageFreezeTrigger'
      | sbobj.Groups.Signals(14).XData = [0 10]
      | sbobj.Groups.Signals(14).YData = [1 1]
      | sbobj.Groups.Signals(15).Name = 'JumpDownEn'
      | sbobj.Groups.Signals(15).XData = [0 10]
      | sbobj.Groups.Signals(15).YData = [1 1]
  EnableSubsystem : Outport  Tag=STV Outport
  DiagInput : Outport  Tag=STV Outport  Port=2
  StartupComp : Outport  Tag=STV Outport  Port=3
  MaxValue : Outport  Tag=STV Outport  Port=4
  MinValue : Outport  Tag=STV Outport  Port=5
  UpCount : Outport  Tag=STV Outport  Port=6
  DownCount : Outport  Tag=STV Outport  Port=7
  FaultCountThd : Outport  Tag=STV Outport  Port=8
  PassCountThd : Outport  Tag=STV Outport  Port=9
  DebounceEn : Outport  Tag=STV Outport  Port=10
  DiagReset : Outport  Tag=STV Outport  Port=11
  DiagEnable : Outport  Tag=STV Outport  Port=12
  HealEnable : Outport  Tag=STV Outport  Port=13
  PreestorageFreezeTrigger : Outport  Tag=STV Outport  Port=14
  JumpDownEn : Outport  Tag=STV Outport  Port=15
  wires:
  Demux/15 -> JumpDownEn/1
  Demux/14 -> PreestorageFreezeTrigger/1
  Demux/13 -> HealEnable/1
  Demux/12 -> DiagEnable/1
  Demux/11 -> DiagReset/1
  Demux/10 -> DebounceEn/1
  Demux/9 -> PassCountThd/1
  Demux/8 -> FaultCountThd/1
  Demux/7 -> DownCount/1
  Demux/6 -> UpCount/1
  Demux/5 -> MinValue/1
  Demux/4 -> MaxValue/1
  Demux/3 -> StartupComp/1
  Demux/2 -> DiagInput/1
  Demux/1 -> EnableSubsystem/1
  FromWs/1 -> Demux/1

== system DiagCCaller_TestHarness/Debounce Enabled - RESET by Disable\Enable subsystem,Fault Inactive, , FaultCnt = 10, PassCnt = 0 , Heal 0 1/Signal Builder ==
  Demux : Demux  Tag=STV Demux  Outputs=15
  FromWs : FromWorkspace  Tag=STV FromWs  VariableName=tuvar  SampleTime=0
      SigBuilderData=|
      | common.afterFinalStr = 'Extrapolate'
      | common.sampleTime = 0
      | dataSet.timeRange = [0 10]
      | dataSet.name = 'Group 1'
      | sbobj.Groups.Name = 'Group 1'
      | sbobj.Groups.Signals(1).Name = 'EnableSubsystem'
      | sbobj.Groups.Signals(1).XData = [0 2.59 2.59 3.42 3.42 4.36 4.94 9.06 9.06 10]
      | sbobj.Groups.Signals(1).YData = [1 1 0 0 1 1 1 1 0 0]
      | sbobj.Groups.Signals(2).Name = 'DiagInput'
      | sbobj.Groups.Signals(2).XData = [0 1 2.41 4.96 4.96 6.23 6.23 6.91 6.91 7.36 7.36 8.36 8.36 9.5 9.5 10]
      | sbobj.Groups.Signals(2).YData = [0 0 0 0 1.1 1.1 0 0 1 1 0 0 1.2 1.2 0 0]
      | sbobj.Groups.Signals(3).Name = 'StartupComp'
      | sbobj.Groups.Signals(3).XData = [0 10]
      | sbobj.Groups.Signals(3).YData = [1 1]
      | sbobj.Groups.Signals(4).Name = 'MaxValue'
      | sbobj.Groups.Signals(4).XData = [0 10]
      | sbobj.Groups.Signals(4).YData = [9999 9999]
      | sbobj.Groups.Signals(5).Name = 'MinValue'
      | sbobj.Groups.Signals(5).XData = [0 10]
      | sbobj.Groups.Signals(5).YData = [-69.9 -69.9]
      | sbobj.Groups.Signals(6).Name = 'UpCount'
      | sbobj.Groups.Signals(6).XData = [0 10]
      | sbobj.Groups.Signals(6).YData = [1 1]
      | sbobj.Groups.Signals(7).Name = 'DownCount'
      | sbobj.Groups.Signals(7).XData = [0 10]
      | sbobj.Groups.Signals(7).YData = [1 1]
      | sbobj.Groups.Signals(8).Name = 'FaultCountThd'
      | sbobj.Groups.Signals(8).XData = [0 10]
      | sbobj.Groups.Signals(8).YData = [10 10]
      | sbobj.Groups.Signals(9).Name = 'PassCountThd'
      | sbobj.Groups.Signals(9).XData = [0 10]
      | sbobj.Groups.Signals(9).YData = [-5 -5]
      | sbobj.Groups.Signals(10).Name = 'DebounceEn'
      | sbobj.Groups.Signals(10).XData = [0 10]
      | sbobj.Groups.Signals(10).YData = [1 1]
      | sbobj.Groups.Signals(11).Name = 'DiagReset'
      | sbobj.Groups.Signals(11).XData = [0 10]
      | sbobj.Groups.Signals(11).YData = [0 0]
      | sbobj.Groups.Signals(12).Name = 'DiagEnable'
      | sbobj.Groups.Signals(12).XData = [0 5.37 5.37 6.72 6.72 10]
      | sbobj.Groups.Signals(12).YData = [1 1 0 0 1 1]
      | sbobj.Groups.Signals(13).Name = 'HealEnable'
      | sbobj.Groups.Signals(13).XData = [0 10]
      | sbobj.Groups.Signals(13).YData = [0 0]
      | sbobj.Groups.Signals(14).Name = 'PreestorageFreezeTrigger'
      | sbobj.Groups.Signals(14).XData = [0 10]
      | sbobj.Groups.Signals(14).YData = [1 1]
      | sbobj.Groups.Signals(15).Name = 'JumpDownEn'
      | sbobj.Groups.Signals(15).XData = [0 10]
      | sbobj.Groups.Signals(15).YData = [1 1]
  EnableSubsystem : Outport  Tag=STV Outport
  DiagInput : Outport  Tag=STV Outport  Port=2
  StartupComp : Outport  Tag=STV Outport  Port=3
  MaxValue : Outport  Tag=STV Outport  Port=4
  MinValue : Outport  Tag=STV Outport  Port=5
  UpCount : Outport  Tag=STV Outport  Port=6
  DownCount : Outport  Tag=STV Outport  Port=7
  FaultCountThd : Outport  Tag=STV Outport  Port=8
  PassCountThd : Outport  Tag=STV Outport  Port=9
  DebounceEn : Outport  Tag=STV Outport  Port=10
  DiagReset : Outport  Tag=STV Outport  Port=11
  DiagEnable : Outport  Tag=STV Outport  Port=12
  HealEnable : Outport  Tag=STV Outport  Port=13
  PreestorageFreezeTrigger : Outport  Tag=STV Outport  Port=14
  JumpDownEn : Outport  Tag=STV Outport  Port=15
  wires:
  FromWs/1 -> Demux/1
  Demux/1 -> EnableSubsystem/1
  Demux/2 -> DiagInput/1
  Demux/3 -> StartupComp/1
  Demux/4 -> MaxValue/1
  Demux/5 -> MinValue/1
  Demux/6 -> UpCount/1
  Demux/7 -> DownCount/1
  Demux/8 -> FaultCountThd/1
  Demux/9 -> PassCountThd/1
  Demux/10 -> DebounceEn/1
  Demux/11 -> DiagReset/1
  Demux/12 -> DiagEnable/1
  Demux/13 -> HealEnable/1
  Demux/14 -> PreestorageFreezeTrigger/1
  Demux/15 -> JumpDownEn/1

== system DiagCCaller_TestHarness/Debounce Enabled - StartUpComp delay = 1s, Fault Active , FaultCnt = 10, PassCnt = -5 , Heal 1 /Signal Builder ==
  Demux : Demux  Tag=STV Demux  Outputs=15
  FromWs : FromWorkspace  Tag=STV FromWs  VariableName=tuvar  SampleTime=0
      SigBuilderData=|
      | common.afterFinalStr = 'Extrapolate'
      | common.sampleTime = 0
      | dataSet.timeRange = [0 10]
      | dataSet.name = 'Group 1'
      | sbobj.Groups.Name = 'Group 1'
      | sbobj.Groups.Signals(1).Name = 'EnableSubsystem'
      | sbobj.Groups.Signals(1).XData = [0 4.36 4.94 9.06 9.06 10]
      | sbobj.Groups.Signals(1).YData = [1 1 1 1 0 0]
      | sbobj.Groups.Signals(2).Name = 'DiagInput'
      | sbobj.Groups.Signals(2).XData = [0 1 1 2.41 2.41 3.88 3.88 6 6 8 8 9.5 9.5 10]
      | sbobj.Groups.Signals(2).YData = [1 1 1 1 0 0 1.1 1.1 0 0 1.2 1.2 0 0]
      | sbobj.Groups.Signals(3).Name = 'StartupComp'
      | sbobj.Groups.Signals(3).XData = [0 1 1 10]
      | sbobj.Groups.Signals(3).YData = [0 0 1 1]
      | sbobj.Groups.Signals(4).Name = 'MaxValue'
      | sbobj.Groups.Signals(4).XData = [0 10]
      | sbobj.Groups.Signals(4).YData = [9999 9999]
      | sbobj.Groups.Signals(5).Name = 'MinValue'
      | sbobj.Groups.Signals(5).XData = [0 10]
      | sbobj.Groups.Signals(5).YData = [-69.9 -69.9]
      | sbobj.Groups.Signals(6).Name = 'UpCount'
      | sbobj.Groups.Signals(6).XData = [0 10]
      | sbobj.Groups.Signals(6).YData = [1 1]
      | sbobj.Groups.Signals(7).Name = 'DownCount'
      | sbobj.Groups.Signals(7).XData = [0 10]
      | sbobj.Groups.Signals(7).YData = [1 1]
      | sbobj.Groups.Signals(8).Name = 'FaultCountThd'
      | sbobj.Groups.Signals(8).XData = [0 10]
      | sbobj.Groups.Signals(8).YData = [10 10]
      | sbobj.Groups.Signals(9).Name = 'PassCountThd'
      | sbobj.Groups.Signals(9).XData = [0 10]
      | sbobj.Groups.Signals(9).YData = [-5 -5]
      | sbobj.Groups.Signals(10).Name = 'DebounceEn'
      | sbobj.Groups.Signals(10).XData = [0 10]
      | sbobj.Groups.Signals(10).YData = [1 1]
      | sbobj.Groups.Signals(11).Name = 'DiagReset'
      | sbobj.Groups.Signals(11).XData = [0 10]
      | sbobj.Groups.Signals(11).YData = [0 0]
      | sbobj.Groups.Signals(12).Name = 'DiagEnable'
      | sbobj.Groups.Signals(12).XData = [0 10]
      | sbobj.Groups.Signals(12).YData = [1 1]
      | sbobj.Groups.Signals(13).Name = 'HealEnable'
      | sbobj.Groups.Signals(13).XData = [0 10]
      | sbobj.Groups.Signals(13).YData = [1 1]
      | sbobj.Groups.Signals(14).Name = 'PreestorageFreezeTrigger'
      | sbobj.Groups.Signals(14).XData = [0 10]
      | sbobj.Groups.Signals(14).YData = [1 1]
      | sbobj.Groups.Signals(15).Name = 'JumpDownEn'
      | sbobj.Groups.Signals(15).XData = [0 10]
      | sbobj.Groups.Signals(15).YData = [0 0]
  EnableSubsystem : Outport  Tag=STV Outport
  DiagInput : Outport  Tag=STV Outport  Port=2
  StartupComp : Outport  Tag=STV Outport  Port=3
  MaxValue : Outport  Tag=STV Outport  Port=4
  MinValue : Outport  Tag=STV Outport  Port=5
  UpCount : Outport  Tag=STV Outport  Port=6
  DownCount : Outport  Tag=STV Outport  Port=7
  FaultCountThd : Outport  Tag=STV Outport  Port=8
  PassCountThd : Outport  Tag=STV Outport  Port=9
  DebounceEn : Outport  Tag=STV Outport  Port=10
  DiagReset : Outport  Tag=STV Outport  Port=11
  DiagEnable : Outport  Tag=STV Outport  Port=12
  HealEnable : Outport  Tag=STV Outport  Port=13
  PreestorageFreezeTrigger : Outport  Tag=STV Outport  Port=14
  JumpDownEn : Outport  Tag=STV Outport  Port=15
  wires:
  FromWs/1 -> Demux/1
  Demux/1 -> EnableSubsystem/1
  Demux/2 -> DiagInput/1
  Demux/3 -> StartupComp/1
  Demux/4 -> MaxValue/1
  Demux/5 -> MinValue/1
  Demux/6 -> UpCount/1
  Demux/7 -> DownCount/1
  Demux/8 -> FaultCountThd/1
  Demux/9 -> PassCountThd/1
  Demux/10 -> DebounceEn/1
  Demux/11 -> DiagReset/1
  Demux/12 -> DiagEnable/1
  Demux/13 -> HealEnable/1
  Demux/14 -> PreestorageFreezeTrigger/1
  Demux/15 -> JumpDownEn/1

== system DiagCCaller_TestHarness/Debounce Enabled - StartUpComp delay = 1s, Fault Active , FaultCnt = 10, PassCnt = 0 , Heal 0 /Signal Builder ==
  Demux : Demux  Tag=STV Demux  Outputs=15
  FromWs : FromWorkspace  Tag=STV FromWs  VariableName=tuvar  SampleTime=0
      SigBuilderData=|
      | common.afterFinalStr = 'Extrapolate'
      | common.sampleTime = 0
      | dataSet.timeRange = [0 10]
      | dataSet.name = 'Group 1'
      | sbobj.Groups.Name = 'Group 1'
      | sbobj.Groups.Signals(1).Name = 'EnableSubsystem'
      | sbobj.Groups.Signals(1).XData = [0 4.36 4.94 9.06 9.06 10]
      | sbobj.Groups.Signals(1).YData = [1 1 1 1 0 0]
      | sbobj.Groups.Signals(2).Name = 'DiagInput'
      | sbobj.Groups.Signals(2).XData = [0 1 1 2.41 2.41 3.88 3.88 6 6 8 8 9.5 9.5 10]
      | sbobj.Groups.Signals(2).YData = [1 1 1 1 0 0 1.1 1.1 0 0 1.2 1.2 0 0]
      | sbobj.Groups.Signals(3).Name = 'StartupComp'
      | sbobj.Groups.Signals(3).XData = [0 1 1 10]
      | sbobj.Groups.Signals(3).YData = [0 0 1 1]
      | sbobj.Groups.Signals(4).Name = 'MaxValue'
      | sbobj.Groups.Signals(4).XData = [0 10]
      | sbobj.Groups.Signals(4).YData = [9999 9999]
      | sbobj.Groups.Signals(5).Name = 'MinValue'
      | sbobj.Groups.Signals(5).XData = [0 10]
      | sbobj.Groups.Signals(5).YData = [-69.9 -69.9]
      | sbobj.Groups.Signals(6).Name = 'UpCount'
      | sbobj.Groups.Signals(6).XData = [0 10]
      | sbobj.Groups.Signals(6).YData = [1 1]
      | sbobj.Groups.Signals(7).Name = 'DownCount'
      | sbobj.Groups.Signals(7).XData = [0 10]
      | sbobj.Groups.Signals(7).YData = [1 1]
      | sbobj.Groups.Signals(8).Name = 'FaultCountThd'
      | sbobj.Groups.Signals(8).XData = [0 10]
      | sbobj.Groups.Signals(8).YData = [10 10]
      | sbobj.Groups.Signals(9).Name = 'PassCountThd'
      | sbobj.Groups.Signals(9).XData = [0 10]
      | sbobj.Groups.Signals(9).YData = [0 0]
      | sbobj.Groups.Signals(10).Name = 'DebounceEn'
      | sbobj.Groups.Signals(10).XData = [0 10]
      | sbobj.Groups.Signals(10).YData = [1 1]
      | sbobj.Groups.Signals(11).Name = 'DiagReset'
      | sbobj.Groups.Signals(11).XData = [0 10]
      | sbobj.Groups.Signals(11).YData = [0 0]
      | sbobj.Groups.Signals(12).Name = 'DiagEnable'
      | sbobj.Groups.Signals(12).XData = [0 10]
      | sbobj.Groups.Signals(12).YData = [1 1]
      | sbobj.Groups.Signals(13).Name = 'HealEnable'
      | sbobj.Groups.Signals(13).XData = [0 10]
      | sbobj.Groups.Signals(13).YData = [0 0]
      | sbobj.Groups.Signals(14).Name = 'PreestorageFreezeTrigger'
      | sbobj.Groups.Signals(14).XData = [0 10]
      | sbobj.Groups.Signals(14).YData = [1 1]
      | sbobj.Groups.Signals(15).Name = 'JumpDownEn'
      | sbobj.Groups.Signals(15).XData = [0 10]
      | sbobj.Groups.Signals(15).YData = [0 0]
  EnableSubsystem : Outport  Tag=STV Outport
  DiagInput : Outport  Tag=STV Outport  Port=2
  StartupComp : Outport  Tag=STV Outport  Port=3
  MaxValue : Outport  Tag=STV Outport  Port=4
  MinValue : Outport  Tag=STV Outport  Port=5
  UpCount : Outport  Tag=STV Outport  Port=6
  DownCount : Outport  Tag=STV Outport  Port=7
  FaultCountThd : Outport  Tag=STV Outport  Port=8
  PassCountThd : Outport  Tag=STV Outport  Port=9
  DebounceEn : Outport  Tag=STV Outport  Port=10
  DiagReset : Outport  Tag=STV Outport  Port=11
  DiagEnable : Outport  Tag=STV Outport  Port=12
  HealEnable : Outport  Tag=STV Outport  Port=13
  PreestorageFreezeTrigger : Outport  Tag=STV Outport  Port=14
  JumpDownEn : Outport  Tag=STV Outport  Port=15
  wires:
  Demux/15 -> JumpDownEn/1
  Demux/14 -> PreestorageFreezeTrigger/1
  Demux/13 -> HealEnable/1
  Demux/12 -> DiagEnable/1
  Demux/11 -> DiagReset/1
  Demux/10 -> DebounceEn/1
  Demux/9 -> PassCountThd/1
  Demux/8 -> FaultCountThd/1
  Demux/7 -> DownCount/1
  Demux/6 -> UpCount/1
  Demux/5 -> MinValue/1
  Demux/4 -> MaxValue/1
  Demux/3 -> StartupComp/1
  Demux/2 -> DiagInput/1
  Demux/1 -> EnableSubsystem/1
  FromWs/1 -> Demux/1

== system DiagCCaller_TestHarness/Debounce Enabled - StartUpComp delay = 1s, Fault Inactive , FaultCnt = 10, PassCnt = -5, Heal 1 /Signal Builder ==
  Demux : Demux  Tag=STV Demux  Outputs=15
  FromWs : FromWorkspace  Tag=STV FromWs  VariableName=tuvar  SampleTime=0
      SigBuilderData=|
      | common.afterFinalStr = 'Extrapolate'
      | common.sampleTime = 0
      | dataSet.timeRange = [0 10]
      | dataSet.name = 'Group 1'
      | sbobj.Groups.Name = 'Group 1'
      | sbobj.Groups.Signals(1).Name = 'EnableSubsystem'
      | sbobj.Groups.Signals(1).XData = [0 4.36 4.94 9.06 9.06 10]
      | sbobj.Groups.Signals(1).YData = [1 1 1 1 0 0]
      | sbobj.Groups.Signals(2).Name = 'DiagInput'
      | sbobj.Groups.Signals(2).XData = [0 1 2.41 3.88 3.88 6 6 8 8 9.5 9.5 10]
      | sbobj.Groups.Signals(2).YData = [0 0 0 0 1.1 1.1 0 0 1.2 1.2 0 0]
      | sbobj.Groups.Signals(3).Name = 'StartupComp'
      | sbobj.Groups.Signals(3).XData = [0 1 1 10]
      | sbobj.Groups.Signals(3).YData = [0 0 1 1]
      | sbobj.Groups.Signals(4).Name = 'MaxValue'
      | sbobj.Groups.Signals(4).XData = [0 10]
      | sbobj.Groups.Signals(4).YData = [9999 9999]
      | sbobj.Groups.Signals(5).Name = 'MinValue'
      | sbobj.Groups.Signals(5).XData = [0 10]
      | sbobj.Groups.Signals(5).YData = [-69.9 -69.9]
      | sbobj.Groups.Signals(6).Name = 'UpCount'
      | sbobj.Groups.Signals(6).XData = [0 10]
      | sbobj.Groups.Signals(6).YData = [1 1]
      | sbobj.Groups.Signals(7).Name = 'DownCount'
      | sbobj.Groups.Signals(7).XData = [0 10]
      | sbobj.Groups.Signals(7).YData = [1 1]
      | sbobj.Groups.Signals(8).Name = 'FaultCountThd'
      | sbobj.Groups.Signals(8).XData = [0 10]
      | sbobj.Groups.Signals(8).YData = [10 10]
      | sbobj.Groups.Signals(9).Name = 'PassCountThd'
      | sbobj.Groups.Signals(9).XData = [0 10]
      | sbobj.Groups.Signals(9).YData = [-5 -5]
      | sbobj.Groups.Signals(10).Name = 'DebounceEn'
      | sbobj.Groups.Signals(10).XData = [0 10]
      | sbobj.Groups.Signals(10).YData = [1 1]
      | sbobj.Groups.Signals(11).Name = 'DiagReset'
      | sbobj.Groups.Signals(11).XData = [0 10]
      | sbobj.Groups.Signals(11).YData = [0 0]
      | sbobj.Groups.Signals(12).Name = 'DiagEnable'
      | sbobj.Groups.Signals(12).XData = [0 10]
      | sbobj.Groups.Signals(12).YData = [1 1]
      | sbobj.Groups.Signals(13).Name = 'HealEnable'
      | sbobj.Groups.Signals(13).XData = [0 10]
      | sbobj.Groups.Signals(13).YData = [1 1]
      | sbobj.Groups.Signals(14).Name = 'PreestorageFreezeTrigger'
      | sbobj.Groups.Signals(14).XData = [0 10]
      | sbobj.Groups.Signals(14).YData = [1 1]
      | sbobj.Groups.Signals(15).Name = 'JumpDownEn'
      | sbobj.Groups.Signals(15).XData = [0 10]
      | sbobj.Groups.Signals(15).YData = [0 0]
  EnableSubsystem : Outport  Tag=STV Outport
  DiagInput : Outport  Tag=STV Outport  Port=2
  StartupComp : Outport  Tag=STV Outport  Port=3
  MaxValue : Outport  Tag=STV Outport  Port=4
  MinValue : Outport  Tag=STV Outport  Port=5
  UpCount : Outport  Tag=STV Outport  Port=6
  DownCount : Outport  Tag=STV Outport  Port=7
  FaultCountThd : Outport  Tag=STV Outport  Port=8
  PassCountThd : Outport  Tag=STV Outport  Port=9
  DebounceEn : Outport  Tag=STV Outport  Port=10
  DiagReset : Outport  Tag=STV Outport  Port=11
  DiagEnable : Outport  Tag=STV Outport  Port=12
  HealEnable : Outport  Tag=STV Outport  Port=13
  PreestorageFreezeTrigger : Outport  Tag=STV Outport  Port=14
  JumpDownEn : Outport  Tag=STV Outport  Port=15
  wires:
  Demux/15 -> JumpDownEn/1
  Demux/14 -> PreestorageFreezeTrigger/1
  Demux/13 -> HealEnable/1
  Demux/12 -> DiagEnable/1
  Demux/11 -> DiagReset/1
  Demux/10 -> DebounceEn/1
  Demux/9 -> PassCountThd/1
  Demux/8 -> FaultCountThd/1
  Demux/7 -> DownCount/1
  Demux/6 -> UpCount/1
  Demux/5 -> MinValue/1
  Demux/4 -> MaxValue/1
  Demux/3 -> StartupComp/1
  Demux/2 -> DiagInput/1
  Demux/1 -> EnableSubsystem/1
  FromWs/1 -> Demux/1

== system DiagCCaller_TestHarness/Debounce Enabled - StartUpComp delay = 1s, Fault Inactive , FaultCnt = 10, PassCnt = 0 , Heal 0 /Signal Builder ==
  Demux : Demux  Tag=STV Demux  Outputs=15
  FromWs : FromWorkspace  Tag=STV FromWs  VariableName=tuvar  SampleTime=0
      SigBuilderData=|
      | common.afterFinalStr = 'Extrapolate'
      | common.sampleTime = 0
      | dataSet.timeRange = [0 10]
      | dataSet.name = 'Group 1'
      | sbobj.Groups.Name = 'Group 1'
      | sbobj.Groups.Signals(1).Name = 'EnableSubsystem'
      | sbobj.Groups.Signals(1).XData = [0 4.36 4.94 9.06 9.06 10]
      | sbobj.Groups.Signals(1).YData = [1 1 1 1 0 0]
      | sbobj.Groups.Signals(2).Name = 'DiagInput'
      | sbobj.Groups.Signals(2).XData = [0 1 2.41 3.88 3.88 6 6 8 8 9.5 9.5 10]
      | sbobj.Groups.Signals(2).YData = [0 0 0 0 1.1 1.1 0 0 1.2 1.2 0 0]
      | sbobj.Groups.Signals(3).Name = 'StartupComp'
      | sbobj.Groups.Signals(3).XData = [0 1 1 10]
      | sbobj.Groups.Signals(3).YData = [0 0 1 1]
      | sbobj.Groups.Signals(4).Name = 'MaxValue'
      | sbobj.Groups.Signals(4).XData = [0 10]
      | sbobj.Groups.Signals(4).YData = [9999 9999]
      | sbobj.Groups.Signals(5).Name = 'MinValue'
      | sbobj.Groups.Signals(5).XData = [0 10]
      | sbobj.Groups.Signals(5).YData = [-69.9 -69.9]
      | sbobj.Groups.Signals(6).Name = 'UpCount'
      | sbobj.Groups.Signals(6).XData = [0 10]
      | sbobj.Groups.Signals(6).YData = [1 1]
      | sbobj.Groups.Signals(7).Name = 'DownCount'
      | sbobj.Groups.Signals(7).XData = [0 10]
      | sbobj.Groups.Signals(7).YData = [1 1]
      | sbobj.Groups.Signals(8).Name = 'FaultCountThd'
      | sbobj.Groups.Signals(8).XData = [0 10]
      | sbobj.Groups.Signals(8).YData = [10 10]
      | sbobj.Groups.Signals(9).Name = 'PassCountThd'
      | sbobj.Groups.Signals(9).XData = [0 10]
      | sbobj.Groups.Signals(9).YData = [0 0]
      | sbobj.Groups.Signals(10).Name = 'DebounceEn'
      | sbobj.Groups.Signals(10).XData = [0 10]
      | sbobj.Groups.Signals(10).YData = [1 1]
      | sbobj.Groups.Signals(11).Name = 'DiagReset'
      | sbobj.Groups.Signals(11).XData = [0 10]
      | sbobj.Groups.Signals(11).YData = [0 0]
      | sbobj.Groups.Signals(12).Name = 'DiagEnable'
      | sbobj.Groups.Signals(12).XData = [0 10]
      | sbobj.Groups.Signals(12).YData = [1 1]
      | sbobj.Groups.Signals(13).Name = 'HealEnable'
      | sbobj.Groups.Signals(13).XData = [0 10]
      | sbobj.Groups.Signals(13).YData = [0 0]
      | sbobj.Groups.Signals(14).Name = 'PreestorageFreezeTrigger'
      | sbobj.Groups.Signals(14).XData = [0 10]
      | sbobj.Groups.Signals(14).YData = [1 1]
      | sbobj.Groups.Signals(15).Name = 'JumpDownEn'
      | sbobj.Groups.Signals(15).XData = [0 10]
      | sbobj.Groups.Signals(15).YData = [1 1]
  EnableSubsystem : Outport  Tag=STV Outport
  DiagInput : Outport  Tag=STV Outport  Port=2
  StartupComp : Outport  Tag=STV Outport  Port=3
  MaxValue : Outport  Tag=STV Outport  Port=4
  MinValue : Outport  Tag=STV Outport  Port=5
  UpCount : Outport  Tag=STV Outport  Port=6
  DownCount : Outport  Tag=STV Outport  Port=7
  FaultCountThd : Outport  Tag=STV Outport  Port=8
  PassCountThd : Outport  Tag=STV Outport  Port=9
  DebounceEn : Outport  Tag=STV Outport  Port=10
  DiagReset : Outport  Tag=STV Outport  Port=11
  DiagEnable : Outport  Tag=STV Outport  Port=12
  HealEnable : Outport  Tag=STV Outport  Port=13
  PreestorageFreezeTrigger : Outport  Tag=STV Outport  Port=14
  JumpDownEn : Outport  Tag=STV Outport  Port=15
  wires:
  FromWs/1 -> Demux/1
  Demux/1 -> EnableSubsystem/1
  Demux/2 -> DiagInput/1
  Demux/3 -> StartupComp/1
  Demux/4 -> MaxValue/1
  Demux/5 -> MinValue/1
  Demux/6 -> UpCount/1
  Demux/7 -> DownCount/1
  Demux/8 -> FaultCountThd/1
  Demux/9 -> PassCountThd/1
  Demux/10 -> DebounceEn/1
  Demux/11 -> DiagReset/1
  Demux/12 -> DiagEnable/1
  Demux/13 -> HealEnable/1
  Demux/14 -> PreestorageFreezeTrigger/1
  Demux/15 -> JumpDownEn/1

== system DiagCCaller_TestHarness/DebounceDisabled - RESET by Calibration DiagReset /Signal Builder ==
  Demux : Demux  Tag=STV Demux  Outputs=15
  FromWs : FromWorkspace  Tag=STV FromWs  VariableName=tuvar  SampleTime=0
      SigBuilderData=|
      | common.afterFinalStr = 'Extrapolate'
      | common.sampleTime = 0
      | dataSet.timeRange = [0 10]
      | dataSet.name = 'Group 1'
      | sbobj.Groups.Name = 'Group 1'
      | sbobj.Groups.Signals(1).Name = 'EnableSubsystem'
      | sbobj.Groups.Signals(1).XData = [0 4.36 4.94 9.06 9.06 10]
      | sbobj.Groups.Signals(1).YData = [1 1 1 1 0 0]
      | sbobj.Groups.Signals(2).Name = 'DiagInput'
      | sbobj.Groups.Signals(2).XData = [0 1 1 2.41 2.41 3.88 3.88 6 6 8 8 9.5 9.5 10]
      | sbobj.Groups.Signals(2).YData = [0 0 1 1 0 0 1.1 1.1 0 0 1.2 1.2 0 0]
      | sbobj.Groups.Signals(3).Name = 'StartupComp'
      | sbobj.Groups.Signals(3).XData = [0 10]
      | sbobj.Groups.Signals(3).YData = [1 1]
      | sbobj.Groups.Signals(4).Name = 'MaxValue'
      | sbobj.Groups.Signals(4).XData = [0 10]
      | sbobj.Groups.Signals(4).YData = [9999 9999]
      | sbobj.Groups.Signals(5).Name = 'MinValue'
      | sbobj.Groups.Signals(5).XData = [0 10]
      | sbobj.Groups.Signals(5).YData = [-69.9 -69.9]
      | sbobj.Groups.Signals(6).Name = 'UpCount'
      | sbobj.Groups.Signals(6).XData = [0 10]
      | sbobj.Groups.Signals(6).YData = [1 1]
      | sbobj.Groups.Signals(7).Name = 'DownCount'
      | sbobj.Groups.Signals(7).XData = [0 10]
      | sbobj.Groups.Signals(7).YData = [1 1]
      | sbobj.Groups.Signals(8).Name = 'FaultCountThd'
      | sbobj.Groups.Signals(8).XData = [0 10]
      | sbobj.Groups.Signals(8).YData = [10 10]
      | sbobj.Groups.Signals(9).Name = 'PassCountThd'
      | sbobj.Groups.Signals(9).XData = [0 10]
      | sbobj.Groups.Signals(9).YData = [0 0]
      | sbobj.Groups.Signals(10).Name = 'DebounceEn'
      | sbobj.Groups.Signals(10).XData = [0 10]
      | sbobj.Groups.Signals(10).YData = [0 0]
      | sbobj.Groups.Signals(11).Name = 'DiagReset'
      | sbobj.Groups.Signals(11).XData = [0 3.42 3.42 5.24 5.24 10]
      | sbobj.Groups.Signals(11).YData = [0 0 1 1 0 0]
      | sbobj.Groups.Signals(12).Name = 'DiagEnable'
      | sbobj.Groups.Signals(12).XData = [0 10]
      | sbobj.Groups.Signals(12).YData = [1 1]
      | sbobj.Groups.Signals(13).Name = 'HealEnable'
      | sbobj.Groups.Signals(13).XData = [0 10]
      | sbobj.Groups.Signals(13).YData = [0 0]
      | sbobj.Groups.Signals(14).Name = 'PreestorageFreezeTrigger'
      | sbobj.Groups.Signals(14).XData = [0 10]
      | sbobj.Groups.Signals(14).YData = [1 1]
      | sbobj.Groups.Signals(15).Name = 'JumpDownEn'
      | sbobj.Groups.Signals(15).XData = [0 10]
      | sbobj.Groups.Signals(15).YData = [1 1]
  EnableSubsystem : Outport  Tag=STV Outport
  DiagInput : Outport  Tag=STV Outport  Port=2
  StartupComp : Outport  Tag=STV Outport  Port=3
  MaxValue : Outport  Tag=STV Outport  Port=4
  MinValue : Outport  Tag=STV Outport  Port=5
  UpCount : Outport  Tag=STV Outport  Port=6
  DownCount : Outport  Tag=STV Outport  Port=7
  FaultCountThd : Outport  Tag=STV Outport  Port=8
  PassCountThd : Outport  Tag=STV Outport  Port=9
  DebounceEn : Outport  Tag=STV Outport  Port=10
  DiagReset : Outport  Tag=STV Outport  Port=11
  DiagEnable : Outport  Tag=STV Outport  Port=12
  HealEnable : Outport  Tag=STV Outport  Port=13
  PreestorageFreezeTrigger : Outport  Tag=STV Outport  Port=14
  JumpDownEn : Outport  Tag=STV Outport  Port=15
  wires:
  Demux/15 -> JumpDownEn/1
  Demux/14 -> PreestorageFreezeTrigger/1
  Demux/13 -> HealEnable/1
  Demux/12 -> DiagEnable/1
  Demux/11 -> DiagReset/1
  Demux/10 -> DebounceEn/1
  Demux/9 -> PassCountThd/1
  Demux/8 -> FaultCountThd/1
  Demux/7 -> DownCount/1
  Demux/6 -> UpCount/1
  Demux/5 -> MinValue/1
  Demux/4 -> MaxValue/1
  Demux/3 -> StartupComp/1
  Demux/2 -> DiagInput/1
  Demux/1 -> EnableSubsystem/1
  FromWs/1 -> Demux/1

== system DiagCCaller_TestHarness/DebounceDisabled - RESET by Disable\Enable subsystem /Signal Builder ==
  Demux : Demux  Tag=STV Demux  Outputs=15
  FromWs : FromWorkspace  Tag=STV FromWs  VariableName=tuvar  SampleTime=0
      SigBuilderData=|
      | common.afterFinalStr = 'Extrapolate'
      | common.sampleTime = 0
      | dataSet.timeRange = [0 10]
      | dataSet.name = 'Group 1'
      | sbobj.Groups.Name = 'Group 1'
      | sbobj.Groups.Signals(1).Name = 'EnableSubsystem'
      | sbobj.Groups.Signals(1).XData = [0 3.12 3.12 4.94 4.94 6.68 6.68 7.7 7.7 9.06 9.06 10]
      | sbobj.Groups.Signals(1).YData = [1 1 0 0 1 1 0 0 1 1 0 0]
      | sbobj.Groups.Signals(2).Name = 'DiagInput'
      | sbobj.Groups.Signals(2).XData = [0 1 2.41 2.41 4.19 4.19 7.46 7.46 9.5 9.5 10]
      | sbobj.Groups.Signals(2).YData = [0 0 0 1.1 1.1 0 0 1.2 1.2 0 0]
      | sbobj.Groups.Signals(3).Name = 'StartupComp'
      | sbobj.Groups.Signals(3).XData = [0 10]
      | sbobj.Groups.Signals(3).YData = [1 1]
      | sbobj.Groups.Signals(4).Name = 'MaxValue'
      | sbobj.Groups.Signals(4).XData = [0 10]
      | sbobj.Groups.Signals(4).YData = [9999 9999]
      | sbobj.Groups.Signals(5).Name = 'MinValue'
      | sbobj.Groups.Signals(5).XData = [0 10]
      | sbobj.Groups.Signals(5).YData = [-69.9 -69.9]
      | sbobj.Groups.Signals(6).Name = 'UpCount'
      | sbobj.Groups.Signals(6).XData = [0 10]
      | sbobj.Groups.Signals(6).YData = [1 1]
      | sbobj.Groups.Signals(7).Name = 'DownCount'
      | sbobj.Groups.Signals(7).XData = [0 10]
      | sbobj.Groups.Signals(7).YData = [1 1]
      | sbobj.Groups.Signals(8).Name = 'FaultCountThd'
      | sbobj.Groups.Signals(8).XData = [0 10]
      | sbobj.Groups.Signals(8).YData = [10 10]
      | sbobj.Groups.Signals(9).Name = 'PassCountThd'
      | sbobj.Groups.Signals(9).XData = [0 10]
      | sbobj.Groups.Signals(9).YData = [0 0]
      | sbobj.Groups.Signals(10).Name = 'DebounceEn'
      | sbobj.Groups.Signals(10).XData = [0 10]
      | sbobj.Groups.Signals(10).YData = [0 0]
      | sbobj.Groups.Signals(11).Name = 'DiagReset'
      | sbobj.Groups.Signals(11).XData = [0 10]
      | sbobj.Groups.Signals(11).YData = [0 0]
      | sbobj.Groups.Signals(12).Name = 'DiagEnable'
      | sbobj.Groups.Signals(12).XData = [0 10]
      | sbobj.Groups.Signals(12).YData = [1 1]
      | sbobj.Groups.Signals(13).Name = 'HealEnable'
      | sbobj.Groups.Signals(13).XData = [0 10]
      | sbobj.Groups.Signals(13).YData = [0 0]
      | sbobj.Groups.Signals(14).Name = 'PreestorageFreezeTrigger'
      | sbobj.Groups.Signals(14).XData = [0 10]
      | sbobj.Groups.Signals(14).YData = [1 1]
      | sbobj.Groups.Signals(15).Name = 'JumpDownEn'
      | sbobj.Groups.Signals(15).XData = [0 10]
      | sbobj.Groups.Signals(15).YData = [1 1]
  EnableSubsystem : Outport  Tag=STV Outport
  DiagInput : Outport  Tag=STV Outport  Port=2
  StartupComp : Outport  Tag=STV Outport  Port=3
  MaxValue : Outport  Tag=STV Outport  Port=4
  MinValue : Outport  Tag=STV Outport  Port=5
  UpCount : Outport  Tag=STV Outport  Port=6
  DownCount : Outport  Tag=STV Outport  Port=7
  FaultCountThd : Outport  Tag=STV Outport  Port=8
  PassCountThd : Outport  Tag=STV Outport  Port=9
  DebounceEn : Outport  Tag=STV Outport  Port=10
  DiagReset : Outport  Tag=STV Outport  Port=11
  DiagEnable : Outport  Tag=STV Outport  Port=12
  HealEnable : Outport  Tag=STV Outport  Port=13
  PreestorageFreezeTrigger : Outport  Tag=STV Outport  Port=14
  JumpDownEn : Outport  Tag=STV Outport  Port=15
  wires:
  Demux/15 -> JumpDownEn/1
  Demux/14 -> PreestorageFreezeTrigger/1
  Demux/13 -> HealEnable/1
  Demux/12 -> DiagEnable/1
  Demux/11 -> DiagReset/1
  Demux/10 -> DebounceEn/1
  Demux/9 -> PassCountThd/1
  Demux/8 -> FaultCountThd/1
  Demux/7 -> DownCount/1
  Demux/6 -> UpCount/1
  Demux/5 -> MinValue/1
  Demux/4 -> MaxValue/1
  Demux/3 -> StartupComp/1
  Demux/2 -> DiagInput/1
  Demux/1 -> EnableSubsystem/1
  FromWs/1 -> Demux/1

== system DiagCCaller_TestHarness/DebounceDisabled INIT Fault Active /Signal Builder ==
  Demux : Demux  Tag=STV Demux  Outputs=15
  FromWs : FromWorkspace  Tag=STV FromWs  VariableName=tuvar  SampleTime=0
      SigBuilderData=|
      | common.afterFinalStr = 'Extrapolate'
      | common.sampleTime = 0
      | dataSet.timeRange = [0 10]
      | dataSet.name = 'Group 1'
      | sbobj.Groups.Name = 'Group 1'
      | sbobj.Groups.Signals(1).Name = 'EnableSubsystem'
      | sbobj.Groups.Signals(1).XData = [0 4.36 4.94 9.06 9.06 10]
      | sbobj.Groups.Signals(1).YData = [1 1 1 1 0 0]
      | sbobj.Groups.Signals(2).Name = 'DiagInput'
      | sbobj.Groups.Signals(2).XData = [0 1 1 2.41 2.41 3.88 3.88 6 6 8 8 9.5 9.5 10]
      | sbobj.Groups.Signals(2).YData = [1 1 1 1 0 0 1.1 1.1 0 0 1.2 1.2 0 0]
      | sbobj.Groups.Signals(3).Name = 'StartupComp'
      | sbobj.Groups.Signals(3).XData = [0 10]
      | sbobj.Groups.Signals(3).YData = [1 1]
      | sbobj.Groups.Signals(4).Name = 'MaxValue'
      | sbobj.Groups.Signals(4).XData = [0 10]
      | sbobj.Groups.Signals(4).YData = [9999 9999]
      | sbobj.Groups.Signals(5).Name = 'MinValue'
      | sbobj.Groups.Signals(5).XData = [0 10]
      | sbobj.Groups.Signals(5).YData = [-69.9 -69.9]
      | sbobj.Groups.Signals(6).Name = 'UpCount'
      | sbobj.Groups.Signals(6).XData = [0 10]
      | sbobj.Groups.Signals(6).YData = [1 1]
      | sbobj.Groups.Signals(7).Name = 'DownCount'
      | sbobj.Groups.Signals(7).XData = [0 10]
      | sbobj.Groups.Signals(7).YData = [1 1]
      | sbobj.Groups.Signals(8).Name = 'FaultCountThd'
      | sbobj.Groups.Signals(8).XData = [0 10]
      | sbobj.Groups.Signals(8).YData = [10 10]
      | sbobj.Groups.Signals(9).Name = 'PassCountThd'
      | sbobj.Groups.Signals(9).XData = [0 10]
      | sbobj.Groups.Signals(9).YData = [0 0]
      | sbobj.Groups.Signals(10).Name = 'DebounceEn'
      | sbobj.Groups.Signals(10).XData = [0 10]
      | sbobj.Groups.Signals(10).YData = [0 0]
      | sbobj.Groups.Signals(11).Name = 'DiagReset'
      | sbobj.Groups.Signals(11).XData = [0 10]
      | sbobj.Groups.Signals(11).YData = [0 0]
      | sbobj.Groups.Signals(12).Name = 'DiagEnable'
      | sbobj.Groups.Signals(12).XData = [0 10]
      | sbobj.Groups.Signals(12).YData = [1 1]
      | sbobj.Groups.Signals(13).Name = 'HealEnable'
      | sbobj.Groups.Signals(13).XData = [0 10]
      | sbobj.Groups.Signals(13).YData = [0 0]
      | sbobj.Groups.Signals(14).Name = 'PreestorageFreezeTrigger'
      | sbobj.Groups.Signals(14).XData = [0 10]
      | sbobj.Groups.Signals(14).YData = [1 1]
      | sbobj.Groups.Signals(15).Name = 'JumpDownEn'
      | sbobj.Groups.Signals(15).XData = [0 10]
      | sbobj.Groups.Signals(15).YData = [1 1]
  EnableSubsystem : Outport  Tag=STV Outport
  DiagInput : Outport  Tag=STV Outport  Port=2
  StartupComp : Outport  Tag=STV Outport  Port=3
  MaxValue : Outport  Tag=STV Outport  Port=4
  MinValue : Outport  Tag=STV Outport  Port=5
  UpCount : Outport  Tag=STV Outport  Port=6
  DownCount : Outport  Tag=STV Outport  Port=7
  FaultCountThd : Outport  Tag=STV Outport  Port=8
  PassCountThd : Outport  Tag=STV Outport  Port=9
  DebounceEn : Outport  Tag=STV Outport  Port=10
  DiagReset : Outport  Tag=STV Outport  Port=11
  DiagEnable : Outport  Tag=STV Outport  Port=12
  HealEnable : Outport  Tag=STV Outport  Port=13
  PreestorageFreezeTrigger : Outport  Tag=STV Outport  Port=14
  JumpDownEn : Outport  Tag=STV Outport  Port=15
  wires:
  Demux/15 -> JumpDownEn/1
  Demux/14 -> PreestorageFreezeTrigger/1
  Demux/13 -> HealEnable/1
  Demux/12 -> DiagEnable/1
  Demux/11 -> DiagReset/1
  Demux/10 -> DebounceEn/1
  Demux/9 -> PassCountThd/1
  Demux/8 -> FaultCountThd/1
  Demux/7 -> DownCount/1
  Demux/6 -> UpCount/1
  Demux/5 -> MinValue/1
  Demux/4 -> MaxValue/1
  Demux/3 -> StartupComp/1
  Demux/2 -> DiagInput/1
  Demux/1 -> EnableSubsystem/1
  FromWs/1 -> Demux/1

== system DiagCCaller_TestHarness/DebounceDisabled INIT Fault Inactive /Signal Builder ==
  Demux : Demux  Tag=STV Demux  Outputs=15
  FromWs : FromWorkspace  Tag=STV FromWs  VariableName=tuvar  SampleTime=0
      SigBuilderData=|
      | common.afterFinalStr = 'Extrapolate'
      | common.sampleTime = 0
      | dataSet.timeRange = [0 10]
      | dataSet.name = 'Group 1'
      | sbobj.Groups.Name = 'Group 1'
      | sbobj.Groups.Signals(1).Name = 'EnableSubsystem'
      | sbobj.Groups.Signals(1).XData = [0 4.36 4.94 9.06 9.06 10]
      | sbobj.Groups.Signals(1).YData = [1 1 1 1 0 0]
      | sbobj.Groups.Signals(2).Name = 'DiagInput'
      | sbobj.Groups.Signals(2).XData = [0 1 2.41 3.88 3.88 6 6 8 8 9.5 9.5 10]
      | sbobj.Groups.Signals(2).YData = [0 0 0 0 1.1 1.1 0 0 1.2 1.2 0 0]
      | sbobj.Groups.Signals(3).Name = 'StartupComp'
      | sbobj.Groups.Signals(3).XData = [0 10]
      | sbobj.Groups.Signals(3).YData = [1 1]
      | sbobj.Groups.Signals(4).Name = 'MaxValue'
      | sbobj.Groups.Signals(4).XData = [0 10]
      | sbobj.Groups.Signals(4).YData = [9999 9999]
      | sbobj.Groups.Signals(5).Name = 'MinValue'
      | sbobj.Groups.Signals(5).XData = [0 10]
      | sbobj.Groups.Signals(5).YData = [-69.9 -69.9]
      | sbobj.Groups.Signals(6).Name = 'UpCount'
      | sbobj.Groups.Signals(6).XData = [0 10]
      | sbobj.Groups.Signals(6).YData = [1 1]
      | sbobj.Groups.Signals(7).Name = 'DownCount'
      | sbobj.Groups.Signals(7).XData = [0 10]
      | sbobj.Groups.Signals(7).YData = [1 1]
      | sbobj.Groups.Signals(8).Name = 'FaultCountThd'
      | sbobj.Groups.Signals(8).XData = [0 10]
      | sbobj.Groups.Signals(8).YData = [10 10]
      | sbobj.Groups.Signals(9).Name = 'PassCountThd'
      | sbobj.Groups.Signals(9).XData = [0 10]
      | sbobj.Groups.Signals(9).YData = [0 0]
      | sbobj.Groups.Signals(10).Name = 'DebounceEn'
      | sbobj.Groups.Signals(10).XData = [0 10]
      | sbobj.Groups.Signals(10).YData = [0 0]
      | sbobj.Groups.Signals(11).Name = 'DiagReset'
      | sbobj.Groups.Signals(11).XData = [0 10]
      | sbobj.Groups.Signals(11).YData = [0 0]
      | sbobj.Groups.Signals(12).Name = 'DiagEnable'
      | sbobj.Groups.Signals(12).XData = [0 10]
      | sbobj.Groups.Signals(12).YData = [1 1]
      | sbobj.Groups.Signals(13).Name = 'HealEnable'
      | sbobj.Groups.Signals(13).XData = [0 10]
      | sbobj.Groups.Signals(13).YData = [0 0]
      | sbobj.Groups.Signals(14).Name = 'PreestorageFreezeTrigger'
      | sbobj.Groups.Signals(14).XData = [0 10]
      | sbobj.Groups.Signals(14).YData = [1 1]
      | sbobj.Groups.Signals(15).Name = 'JumpDownEn'
      | sbobj.Groups.Signals(15).XData = [0 10]
      | sbobj.Groups.Signals(15).YData = [1 1]
  EnableSubsystem : Outport  Tag=STV Outport
  DiagInput : Outport  Tag=STV Outport  Port=2
  StartupComp : Outport  Tag=STV Outport  Port=3
  MaxValue : Outport  Tag=STV Outport  Port=4
  MinValue : Outport  Tag=STV Outport  Port=5
  UpCount : Outport  Tag=STV Outport  Port=6
  DownCount : Outport  Tag=STV Outport  Port=7
  FaultCountThd : Outport  Tag=STV Outport  Port=8
  PassCountThd : Outport  Tag=STV Outport  Port=9
  DebounceEn : Outport  Tag=STV Outport  Port=10
  DiagReset : Outport  Tag=STV Outport  Port=11
  DiagEnable : Outport  Tag=STV Outport  Port=12
  HealEnable : Outport  Tag=STV Outport  Port=13
  PreestorageFreezeTrigger : Outport  Tag=STV Outport  Port=14
  JumpDownEn : Outport  Tag=STV Outport  Port=15
  wires:
  FromWs/1 -> Demux/1
  Demux/1 -> EnableSubsystem/1
  Demux/2 -> DiagInput/1
  Demux/3 -> StartupComp/1
  Demux/4 -> MaxValue/1
  Demux/5 -> MinValue/1
  Demux/6 -> UpCount/1
  Demux/7 -> DownCount/1
  Demux/8 -> FaultCountThd/1
  Demux/9 -> PassCountThd/1
  Demux/10 -> DebounceEn/1
  Demux/11 -> DiagReset/1
  Demux/12 -> DiagEnable/1
  Demux/13 -> HealEnable/1
  Demux/14 -> PreestorageFreezeTrigger/1
  Demux/15 -> JumpDownEn/1

== system DiagCCaller_TestHarness/DebounceDisabled StartUpComp delay = 1s /Signal Builder ==
  Demux : Demux  Tag=STV Demux  Outputs=15
  FromWs : FromWorkspace  Tag=STV FromWs  VariableName=tuvar  SampleTime=0
      SigBuilderData=|
      | common.afterFinalStr = 'Extrapolate'
      | common.sampleTime = 0
      | dataSet.timeRange = [0 10]
      | dataSet.name = 'Group 1'
      | sbobj.Groups.Name = 'Group 1'
      | sbobj.Groups.Signals(1).Name = 'EnableSubsystem'
      | sbobj.Groups.Signals(1).XData = [0 4.36 4.94 9.06 9.06 10]
      | sbobj.Groups.Signals(1).YData = [1 1 1 1 0 0]
      | sbobj.Groups.Signals(2).Name = 'DiagInput'
      | sbobj.Groups.Signals(2).XData = [0 1 2.41 3.88 3.88 6 6 8 8 9.5 9.5 10]
      | sbobj.Groups.Signals(2).YData = [0 0 0 0 1.1 1.1 0 0 1.2 1.2 0 0]
      | sbobj.Groups.Signals(3).Name = 'StartupComp'
      | sbobj.Groups.Signals(3).XData = [0 1 1 10]
      | sbobj.Groups.Signals(3).YData = [0 0 1 1]
      | sbobj.Groups.Signals(4).Name = 'MaxValue'
      | sbobj.Groups.Signals(4).XData = [0 10]
      | sbobj.Groups.Signals(4).YData = [9999 9999]
      | sbobj.Groups.Signals(5).Name = 'MinValue'
      | sbobj.Groups.Signals(5).XData = [0 10]
      | sbobj.Groups.Signals(5).YData = [-69.9 -69.9]
      | sbobj.Groups.Signals(6).Name = 'UpCount'
      | sbobj.Groups.Signals(6).XData = [0 10]
      | sbobj.Groups.Signals(6).YData = [1 1]
      | sbobj.Groups.Signals(7).Name = 'DownCount'
      | sbobj.Groups.Signals(7).XData = [0 10]
      | sbobj.Groups.Signals(7).YData = [1 1]
      | sbobj.Groups.Signals(8).Name = 'FaultCountThd'
      | sbobj.Groups.Signals(8).XData = [0 10]
      | sbobj.Groups.Signals(8).YData = [10 10]
      | sbobj.Groups.Signals(9).Name = 'PassCountThd'
      | sbobj.Groups.Signals(9).XData = [0 10]
      | sbobj.Groups.Signals(9).YData = [0 0]
      | sbobj.Groups.Signals(10).Name = 'DebounceEn'
      | sbobj.Groups.Signals(10).XData = [0 10]
      | sbobj.Groups.Signals(10).YData = [0 0]
      | sbobj.Groups.Signals(11).Name = 'DiagReset'
      | sbobj.Groups.Signals(11).XData = [0 10]
      | sbobj.Groups.Signals(11).YData = [0 0]
      | sbobj.Groups.Signals(12).Name = 'DiagEnable'
      | sbobj.Groups.Signals(12).XData = [0 10]
      | sbobj.Groups.Signals(12).YData = [1 1]
      | sbobj.Groups.Signals(13).Name = 'HealEnable'
      | sbobj.Groups.Signals(13).XData = [0 10]
      | sbobj.Groups.Signals(13).YData = [0 0]
      | sbobj.Groups.Signals(14).Name = 'PreestorageFreezeTrigger'
      | sbobj.Groups.Signals(14).XData = [0 10]
      | sbobj.Groups.Signals(14).YData = [1 1]
      | sbobj.Groups.Signals(15).Name = 'JumpDownEn'
      | sbobj.Groups.Signals(15).XData = [0 10]
      | sbobj.Groups.Signals(15).YData = [1 1]
  EnableSubsystem : Outport  Tag=STV Outport
  DiagInput : Outport  Tag=STV Outport  Port=2
  StartupComp : Outport  Tag=STV Outport  Port=3
  MaxValue : Outport  Tag=STV Outport  Port=4
  MinValue : Outport  Tag=STV Outport  Port=5
  UpCount : Outport  Tag=STV Outport  Port=6
  DownCount : Outport  Tag=STV Outport  Port=7
  FaultCountThd : Outport  Tag=STV Outport  Port=8
  PassCountThd : Outport  Tag=STV Outport  Port=9
  DebounceEn : Outport  Tag=STV Outport  Port=10
  DiagReset : Outport  Tag=STV Outport  Port=11
  DiagEnable : Outport  Tag=STV Outport  Port=12
  HealEnable : Outport  Tag=STV Outport  Port=13
  PreestorageFreezeTrigger : Outport  Tag=STV Outport  Port=14
  JumpDownEn : Outport  Tag=STV Outport  Port=15
  wires:
  Demux/15 -> JumpDownEn/1
  Demux/14 -> PreestorageFreezeTrigger/1
  Demux/13 -> HealEnable/1
  Demux/12 -> DiagEnable/1
  Demux/11 -> DiagReset/1
  Demux/10 -> DebounceEn/1
  Demux/9 -> PassCountThd/1
  Demux/8 -> FaultCountThd/1
  Demux/7 -> DownCount/1
  Demux/6 -> UpCount/1
  Demux/5 -> MinValue/1
  Demux/4 -> MaxValue/1
  Demux/3 -> StartupComp/1
  Demux/2 -> DiagInput/1
  Demux/1 -> EnableSubsystem/1
  FromWs/1 -> Demux/1

== system DiagCCaller_TestHarness/Fault set and recover , FaultCnt = 10, PassCnt = -5 , Heal =1, JumpDownEn = 0 /Signal Builder ==
  Demux : Demux  Tag=STV Demux  Outputs=15
  FromWs : FromWorkspace  Tag=STV FromWs  VariableName=tuvar  SampleTime=0
      SigBuilderData=|
      | common.afterFinalStr = 'Extrapolate'
      | common.sampleTime = 0
      | dataSet.timeRange = [0 10]
      | dataSet.name = 'Group 1'
      | sbobj.Groups.Name = 'Group 1'
      | sbobj.Groups.Signals(1).Name = 'EnableSubsystem'
      | sbobj.Groups.Signals(1).XData = [0 4.36 4.94 9.06 9.06 10]
      | sbobj.Groups.Signals(1).YData = [1 1 1 1 0 0]
      | sbobj.Groups.Signals(2).Name = 'DiagInput'
      | sbobj.Groups.Signals(2).XData = [0 1 1 3.03 3.03 4.91 4.91 6.65 6.65 10]
      | sbobj.Groups.Signals(2).YData = [0 0 1.1 1.1 0 0 1.2 1.2 0 0]
      | sbobj.Groups.Signals(3).Name = 'StartupComp'
      | sbobj.Groups.Signals(3).XData = [0 10]
      | sbobj.Groups.Signals(3).YData = [1 1]
      | sbobj.Groups.Signals(4).Name = 'MaxValue'
      | sbobj.Groups.Signals(4).XData = [0 10]
      | sbobj.Groups.Signals(4).YData = [9999 9999]
      | sbobj.Groups.Signals(5).Name = 'MinValue'
      | sbobj.Groups.Signals(5).XData = [0 10]
      | sbobj.Groups.Signals(5).YData = [-69.9 -69.9]
      | sbobj.Groups.Signals(6).Name = 'UpCount'
      | sbobj.Groups.Signals(6).XData = [0 10]
      | sbobj.Groups.Signals(6).YData = [1 1]
      | sbobj.Groups.Signals(7).Name = 'DownCount'
      | sbobj.Groups.Signals(7).XData = [0 10]
      | sbobj.Groups.Signals(7).YData = [1 1]
      | sbobj.Groups.Signals(8).Name = 'FaultCountThd'
      | sbobj.Groups.Signals(8).XData = [0 10]
      | sbobj.Groups.Signals(8).YData = [10 10]
      | sbobj.Groups.Signals(9).Name = 'PassCountThd'
      | sbobj.Groups.Signals(9).XData = [0 10]
      | sbobj.Groups.Signals(9).YData = [-5 -5]
      | sbobj.Groups.Signals(10).Name = 'DebounceEn'
      | sbobj.Groups.Signals(10).XData = [0 10]
      | sbobj.Groups.Signals(10).YData = [1 1]
      | sbobj.Groups.Signals(11).Name = 'DiagReset'
      | sbobj.Groups.Signals(11).XData = [0 10]
      | sbobj.Groups.Signals(11).YData = [0 0]
      | sbobj.Groups.Signals(12).Name = 'DiagEnable'
      | sbobj.Groups.Signals(12).XData = [0 10]
      | sbobj.Groups.Signals(12).YData = [1 1]
      | sbobj.Groups.Signals(13).Name = 'HealEnable'
      | sbobj.Groups.Signals(13).XData = [0 10]
      | sbobj.Groups.Signals(13).YData = [1 1]
      | sbobj.Groups.Signals(14).Name = 'PreestorageFreezeTrigger'
      | sbobj.Groups.Signals(14).XData = [0 10]
      | sbobj.Groups.Signals(14).YData = [1 1]
      | sbobj.Groups.Signals(15).Name = 'JumpDownEn'
      | sbobj.Groups.Signals(15).XData = [0 10]
      | sbobj.Groups.Signals(15).YData = [0 0]
  EnableSubsystem : Outport  Tag=STV Outport
  DiagInput : Outport  Tag=STV Outport  Port=2
  StartupComp : Outport  Tag=STV Outport  Port=3
  MaxValue : Outport  Tag=STV Outport  Port=4
  MinValue : Outport  Tag=STV Outport  Port=5
  UpCount : Outport  Tag=STV Outport  Port=6
  DownCount : Outport  Tag=STV Outport  Port=7
  FaultCountThd : Outport  Tag=STV Outport  Port=8
  PassCountThd : Outport  Tag=STV Outport  Port=9
  DebounceEn : Outport  Tag=STV Outport  Port=10
  DiagReset : Outport  Tag=STV Outport  Port=11
  DiagEnable : Outport  Tag=STV Outport  Port=12
  HealEnable : Outport  Tag=STV Outport  Port=13
  PreestorageFreezeTrigger : Outport  Tag=STV Outport  Port=14
  JumpDownEn : Outport  Tag=STV Outport  Port=15
  wires:
  FromWs/1 -> Demux/1
  Demux/1 -> EnableSubsystem/1
  Demux/2 -> DiagInput/1
  Demux/3 -> StartupComp/1
  Demux/4 -> MaxValue/1
  Demux/5 -> MinValue/1
  Demux/6 -> UpCount/1
  Demux/7 -> DownCount/1
  Demux/8 -> FaultCountThd/1
  Demux/9 -> PassCountThd/1
  Demux/10 -> DebounceEn/1
  Demux/11 -> DiagReset/1
  Demux/12 -> DiagEnable/1
  Demux/13 -> HealEnable/1
  Demux/14 -> PreestorageFreezeTrigger/1
  Demux/15 -> JumpDownEn/1

== system DiagCCaller_TestHarness/Subsystem/Fault Debounce Lv1 state Input ==
  diagInput : Inport
  diagStartUpComp : Inport  Port=2
  diagUpCnt : Inport  Port=3
  diagDnCnt : Inport  Port=4
  diagFaultCntThresh : Inport  Port=5
  diagPassCntThresh : Inport  Port=6
  diagDbncEnab : Inport  Port=7
  diagReset : Inport  Port=8
  diagEnable : Inport  Port=9
  diagHealEn : Inport  Port=10
  diagPreestorageEn : Inport  Port=11
  diagJumpDownEn : Inport  Port=12
  Ccaller_DiagLv1 : Subsystem  AncestorBlock=common_lib/Diagnostics/Ccaller_DiagLv1  TreatAsAtomicUnit=on
      settings: RTWSystemCode=Nonreusable function
  diagFaultStatus : Outport  OutputWhenDisabled=reset  InitialOutput=Dem_EventStatusType.DEM_EVENT_STATUS_INIT
  diagPreestorageTrigger : Outport  Port=2  OutputWhenDisabled=reset  InitialOutput=Dem_EventStatusType.DEM_EVENT_STATUS_INIT
  Counter : Outport  Port=3  OutputWhenDisabled=reset  InitialOutput=Dem_EventStatusType.DEM_EVENT_STATUS_INIT
  wires:
  diagReset/1 -> Ccaller_DiagLv1/3(diagReset)
  diagDnCnt/1 -> Ccaller_DiagLv1/9(diagDnCnt)
  diagFaultCntThresh/1 -> Ccaller_DiagLv1/6(diagFaultCntThresh)
  diagPassCntThresh/1 -> Ccaller_DiagLv1/7(diagPassCntThresh)
  diagUpCnt/1 -> Ccaller_DiagLv1/8(diagUpCnt)
  diagStartUpComp/1 -> Ccaller_DiagLv1/2(diagStartUpComp)
  diagDbncEnab/1 -> Ccaller_DiagLv1/5(diagDbncEnable)
  diagHealEn/1 -> Ccaller_DiagLv1/10(diagHealEn)
  diagEnable/1 -> Ccaller_DiagLv1/4(diagEnable)
  diagPreestorageEn/1 -> Ccaller_DiagLv1/11(diagPrestorageEn)
  diagJumpDownEn/1 -> Ccaller_DiagLv1/12(diagJumpDownEn)
  Ccaller_DiagLv1/1(diagFaultStatus) -> diagFaultStatus/1
  Ccaller_DiagLv1/2(diagPrestorageTrigger) -> diagPreestorageTrigger/1
  Ccaller_DiagLv1/3(Counter) -> Counter/1
  diagInput/1 -> Ccaller_DiagLv1/1(diagFaultActive)
